simulink model "Quadcopter_close_loop"  (R2021a)
settings: Solver=ode4  StartTime=0.0  StopTime=87  FixedStep=0.001  RelTol=1e-6
values from neighbouring files (symbols this model uses):
  mean_wind = [2.72 , 1.75, -0.006]    [main_run.m]    (also in main_run_5_1.m; param_est.m = [2.72 , 1.75, .006])
  q = X(7:10)    [EKF_without_wind.m]
  r = linspace(floor(nr*0.01)/nr,1,nr)    [main_run.m]    (also in main_run_5_1.m)
  w1 = w(1)    [EKF_without_wind.m]
  x0 = [0,0,0,1,0,0,0,-P.mean_wind,0,0,0]    [main_run.m]    (also in main_run_5_1.m)
  xref = [1,1,-8,1,0,0,0,-P.mean_wind]    [main_run.m]    (also in main_run_5_1.m)
undefined symbols (not defined in the file or in its folder): HDBK, MIL, Moderate, P, u1, v1
libraries: simulink x1, aerolibwind2 x1
(part 3 of 5)

== matlab function Quadcopter_close_loop/Estimator/Estimator/EKF_quadcopter ==
  data: sensor input; y output; P parameter
function y = EKF_quadcopter(sensor,P)
%% parameters 
ts = 0.01;
m = P.m;
g = P.g;
rho = P.rho;
D = P.D;
A_gr = [0;0;g];
B_i = P.B_i;

param = cell(1,6);
param{1} = A_gr;
param{2} = m;
param{3} = rho;
param{4} = D;
param{5} = ts;
param{6} = B_i;

Q_est = P.Q_est;
R_est = P.R_est;
X0_hat = P.X0_hat;
EKF_P0 = P.EKF_P0;
%% IEKF
    persistent k P_cov X
    if isempty(k)
        k = 1;
        X = zeros(13,1);
        [X,P_cov] = EKF(X0_hat,EKF_P0,Q_est,R_est,param,sensor,k);
    end
    k = k+1;
    
    [X,P_cov] = EKF(X,P_cov,Q_est,R_est,param,sensor,k);
    
quat = X(7:10);  
eul = quat2eul(quat')';
eul([1 3]) = eul([3 1]);
X_est = [X(1:6);eul;X(11:13)];
% Asma: Dynamics states: pos, quaternion, velocity, wind? Rearranged the dynamics so that it goes into contoller correctly 

% X_est=[X(1:3); X(7:10); X(4:6); X(11:13)];

y=X_est;
end

function [X_k1,P_k1] = EKF(X,P,Q,R,param,sensor,iter)
% Performs one loop of the SP-EKF.
% Pre-Observer is of the form:
%   Xhat_dot = f(Xhat) + Fr*L*E*(Y - Yhat)

% Inputs:

%   X = State mean, m_k|k-1 (nx1)
%   P = State covariance, P_k|k-1(nxn)
%   f = State dynamics, xdot = f(x,param)
%   df = 
%   dh =
%   Q = Process Noise Covariance Matrix(nxn)
%   R = Measurement Noise Covariance Matrix (mxm)
%   param = Any parameters for f
%   iter = denotes the the first loop,1=yes,0=no

% Outputs:

%   X_k1 = state at next time step
%   P_k1 = state covariance at next time step

%parameter
A_gr = param{1};
m = param{2};
rho = param{3};
D = param{4};
ts = param{5};
B_i = param{6};
b3=[0;0;1];
%sensor
% Y=[sensor{1};sensor{2};sensor{3}]; %gps+accel+B_b
% w = sensor{4};
% f_c = sensor{5};
gps = sensor(1:3);
accel = sensor(4:6);
w = sensor(7:9);
B_b = sensor(10:12);
f_c = sensor(13);

Y=[gps;accel;B_b];
U={w;f_c}; %w+f_c
%states(13*1)
x_hat=X(1:3);
vr_hat=X(4:6);
q_hat=X(7:10);
d_hat=X(11:13);

q0=q_hat(1);q1=q_hat(2);q2=q_hat(3);q3=q_hat(4);
Ln_32 = [-q1/2, -q2/2, -q3/2;
          q0/2, -q3/2,  q2/2;
          q3/2,  q0/2, -q1/2;
         -q2/2,  q1/2,  q0/2];
%Invariant frame (13x10)
Ln =@(vr_hat)[    eye(3)      zeros(3,3)    zeros(3,1) zeros(3,3);
              zeros(3,3)     hat(vr_hat)     -(1/m)*b3  zeros(3,3);
              zeros(4,3)           Ln_32    zeros(4,1) zeros(4,3);
              zeros(3,3)      zeros(3,3)    zeros(3,1)    eye(3);];
%% time update 
    X_minus_k1 = X; %dim(X)=13x1
    P_minus_k1 = P; %dim(P)=12x12
    N=10;
    for i=1:N
    X_minus_k1 = X_minus_k1 + (ts/N).*f(X,U,param);
    
    q_hat=X_minus_k1(7:10);
    q_hat=q_hat/norm(q_hat);    
    X_minus_k1(7:10)=q_hat; %normalization
    A = df(X_minus_k1,U,param);
    
    P_minus_k1 = P_minus_k1 + (ts/N).*(A*P + P*A' + Ln(vr_hat)*Q*Ln(vr_hat)');
%     P_minus_k1 = P_minus_k1 + (ts/N)*(A*P + P*A' + Q);
    end
    X_k1 = X_minus_k1;
    P_k1 = P_minus_k1;
%% measurement update 
    H= dh(X_minus_k1,U,param);
    L = P_minus_k1*H'*inv(H*P_minus_k1*H' + R);
    X_k1 = X_minus_k1 + L*(Y-h(X_minus_k1,U,param));
    q_hat=X_k1(7:10);
    q_hat=q_hat/norm(q_hat);    
    X_k1(7:10)=q_hat; %normalization
    P_k1 = (eye(13)-L*H)*P_minus_k1;
end
 
function [X_dot] = f(X,U,param)
%states
x=X(1:3);
vr=X(4:6);
q=X(7:10);
d=X(11:13);
%inputs
w=U{1};
f_c=U{2};
%parameters
A_gr = param{1};
m = param{2};
rho = param{3};
D = param{4};
B_i= param{6};
b_3=[0;0;1];
%% system dynamics
f_vr=-(1/2)*rho*D*norm(vr)*vr;
x_dot = quat_v(q,vr,0) + d;
vr_dot = cross(vr,w) + quat_v(q,A_gr,1) - (1/m)*f_c*b_3 + (1/m)*f_vr;
q_dot = (1/2)*quat_multiply(q,[0;w]);
d_dot = [0;0;0];
%% output
X_dot = [x_dot;vr_dot;q_dot;d_dot];
end

function [Y] = h(X,U,param)
%states
x=X(1:3);
vr=X(4:6);
q=X(7:10);
d=X(11:13);
%inputs
w=U{1};
f_c=U{2};
%parameters
A_gr = param{1};
m = param{2};
rho = param{3};
D = param{4};
ts = param{5};
B_i = param{6};
b_3=[0;0;1];
%%
f_vr =-(1/2)*rho*D*norm(vr)*vr;
a = - (1/m)*f_c*b_3 + (1/m)*f_vr;
B_b = quat_v(q,B_i,1);
%% ouputs
Y = [x;a;B_b];
end

function [dfdx] = df(X,U,param)
%states
x=X(1:3);
vr=X(4:6);
vr1=vr(1);vr2=vr(2);vr3=vr(3);
q=X(7:10);
d=X(11:13);
q0=q(1);q1=q(2);q2=q(3);q3=q(4);
%inputs
w=U{1};
w1=w(1);w2=w(2);w3=w(3);
f_c=U{2};
%parameters
A_gr = param{1};
g=A_gr(3);
m = param{2};
rho = param{3};
D = param{4};
B_i= param{6};
b_3=[0;0;1];

D11=D(1,1);D22=D(2,2);D33=D(3,3);

df1dx=zeros(3,3);
df1dvr = [-2*q2^2 - 2*q3^2 + 1,2*q1*q2 - 2*q0*q3,2*q0*q2 + 2*q1*q3;
           2*q0*q3 + 2*q1*q2,-2*q1^2 - 2*q3^2 + 1,2*q2*q3 - 2*q0*q1;
           2*q1*q3 - 2*q0*q2,2*q0*q1 + 2*q2*q3,-2*q1^2 - 2*q2^2+1;];
% df1dqv = [2*q2*vr2 + 2*q3*vr3, 2*q0*vr3 + 2*q1*vr2 - 4*q2*vr1, 2*q1*vr3 - 2*q0*vr2 - 4*q3*vr1;
%           2*q2*vr1 - 4*q1*vr2 - 2*q0*vr3,2*q1*vr1 + 2*q3*vr3, 2*q0*vr1 + 2*q2*vr3 - 4*q3*vr2;
%           2*q0*vr2 - 4*q1*vr3 + 2*q3*vr1, 2*q3*vr2 - 4*q2*vr3 - 2*q0*vr1,2*q1*vr1 + 2*q2*vr2;];
df1dq = [2*q2*vr3 - 2*q3*vr2,            2*q2*vr2 + 2*q3*vr3, 2*q0*vr3 + 2*q1*vr2 - 4*q2*vr1, 2*q1*vr3 - 2*q0*vr2 - 4*q3*vr1;
         2*q3*vr1 - 2*q1*vr3, 2*q2*vr1 - 4*q1*vr2 - 2*q0*vr3,            2*q1*vr1 + 2*q3*vr3, 2*q0*vr1 + 2*q2*vr3 - 4*q3*vr2;
         2*q1*vr2 - 2*q2*vr1, 2*q0*vr2 - 4*q1*vr3 + 2*q3*vr1, 2*q3*vr2 - 4*q2*vr3 - 2*q0*vr1,            2*q1*vr1 + 2*q2*vr2];
df1dd = eye(3);

df2dx = zeros(3,3);
df2dvr =[-(D11*rho*(abs(vr1)^2 + abs(vr2)^2 + abs(vr3)^2)^(1/2))/(2*m) - (D11*rho*vr1*abs(vr1)*sign(vr1))/(2*m*(abs(vr1)^2 + abs(vr2)^2 + abs(vr3)^2)^(1/2)),                                                             w3 - (D11*rho*vr1*abs(vr2)*sign(vr2))/(2*m*(abs(vr1)^2 + abs(vr2)^2 + abs(vr3)^2)^(1/2)),                                                           - w2 - (D11*rho*vr1*abs(vr3)*sign(vr3))/(2*m*(abs(vr1)^2 + abs(vr2)^2 + abs(vr3)^2)^(1/2));
                                                                  - w3 - (D22*rho*vr2*abs(vr1)*sign(vr1))/(2*m*(abs(vr1)^2 + abs(vr2)^2 + abs(vr3)^2)^(1/2)), - (D22*rho*(abs(vr1)^2 + abs(vr2)^2 + abs(vr3)^2)^(1/2))/(2*m) - (D22*rho*vr2*abs(vr2)*sign(vr2))/(2*m*(abs(vr1)^2 + abs(vr2)^2 + abs(vr3)^2)^(1/2)),                                                             w1 - (D22*rho*vr2*abs(vr3)*sign(vr3))/(2*m*(abs(vr1)^2 + abs(vr2)^2 + abs(vr3)^2)^(1/2));
                                                                    w2 - (D33*rho*vr3*abs(vr1)*sign(vr1))/(2*m*(abs(vr1)^2 + abs(vr2)^2 + abs(vr3)^2)^(1/2)),                                                           - w1 - (D33*rho*vr3*abs(vr2)*sign(vr2))/(2*m*(abs(vr1)^2 + abs(vr2)^2 + abs(vr3)^2)^(1/2)), - (D33*rho*(abs(vr1)^2 + abs(vr2)^2 + abs(vr3)^2)^(1/2))/(2*m) - (D33*rho*vr3*abs(vr3)*sign(vr3))/(2*m*(abs(vr1)^2 + abs(vr2)^2 + abs(vr3)^2)^(1/2));];
                               
% df2dqv =[(2*g*(2*q0^2*q3 + 6*q1^2*q3 + 2*q2^2*q3 + 2*q3^3 - q3))/(4*q0^2*q1^2 + 4*q0^2*q2^2 + 4*q0^2*q3^2 + 4*q1^4 + 8*q1^2*q2^2 + 8*q1^2*q3^2 - 4*q1^2 + 4*q2^4 + 8*q2^2*q3^2 - 4*q2^2 + 4*q3^4 - 4*q3^2 + 1) - (2*g*(8*q0^2*q1 + 16*q1^3 + 16*q1*q2^2 + 16*q1*q3^2 - 8*q1)*(2*q0^2*q1*q3 - q0*q2 + 2*q1^3*q3 + 2*q1*q2^2*q3 + 2*q1*q3^3 - q1*q3))/(4*q0^2*q1^2 + 4*q0^2*q2^2 + 4*q0^2*q3^2 + 4*q1^4 + 8*q1^2*q2^2 + 8*q1^2*q3^2 - 4*q1^2 + 4*q2^4 + 8*q2^2*q3^2 - 4*q2^2 + 4*q3^4 - 4*q3^2 + 1)^2,                               - (2*g*(q0 - 4*q1*q2*q3))/(4*q0^2*q1^2 + 4*q0^2*q2^2 + 4*q0^2*q3^2 + 4*q1^4 + 8*q1^2*q2^2 + 8*q1^2*q3^2 - 4*q1^2 + 4*q2^4 + 8*q2^2*q3^2 - 4*q2^2 + 4*q3^4 - 4*q3^2 + 1) - (2*g*(8*q0^2*q2 + 16*q1^2*q2 + 16*q2^3 + 16*q2*q3^2 - 8*q2)*(2*q0^2*q1*q3 - q0*q2 + 2*q1^3*q3 + 2*q1*q2^2*q3 + 2*q1*q3^3 - q1*q3))/(4*q0^2*q1^2 + 4*q0^2*q2^2 + 4*q0^2*q3^2 + 4*q1^4 + 8*q1^2*q2^2 + 8*q1^2*q3^2 - 4*q1^2 + 4*q2^4 + 8*q2^2*q3^2 - 4*q2^2 + 4*q3^4 - 4*q3^2 + 1)^2,            (2*g*(2*q0^2*q1 + 2*q1^3 + 2*q1*q2^2 + 6*q1*q3^2 - q1))/(4*q0^2*q1^2 + 4*q0^2*q2^2 + 4*q0^2*q3^2 + 4*q1^4 + 8*q1^2*q2^2 + 8*q1^2*q3^2 - 4*q1^2 + 4*q2^4 + 8*q2^2*q3^2 - 4*q2^2 + 4*q3^4 - 4*q3^2 + 1) - (2*g*(8*q0^2*q3 + 16*q1^2*q3 + 16*q2^2*q3 + 16*q3^3 - 8*q3)*(2*q0^2*q1*q3 - q0*q2 + 2*q1^3*q3 + 2*q1*q2^2*q3 + 2*q1*q3^3 - q1*q3))/(4*q0^2*q1^2 + 4*q0^2*q2^2 + 4*q0^2*q3^2 + 4*q1^4 + 8*q1^2*q2^2 + 8*q1^2*q3^2 - 4*q1^2 + 4*q2^4 + 8*q2^2*q3^2 - 4*q2^2 + 4*q3^4 - 4*q3^2 + 1)^2;
%                                         (2*g*(q0 + 4*q1*q2*q3))/(4*q0^2*q1^2 + 4*q0^2*q2^2 + 4*q0^2*q3^2 + 4*q1^4 + 8*q1^2*q2^2 + 8*q1^2*q3^2 - 4*q1^2 + 4*q2^4 + 8*q2^2*q3^2 - 4*q2^2 + 4*q3^4 - 4*q3^2 + 1) - (2*g*(8*q0^2*q1 + 16*q1^3 + 16*q1*q2^2 + 16*q1*q3^2 - 8*q1)*(2*q0^2*q2*q3 + q0*q1 + 2*q1^2*q2*q3 + 2*q2^3*q3 + 2*q2*q3^3 - q2*q3))/(4*q0^2*q1^2 + 4*q0^2*q2^2 + 4*q0^2*q3^2 + 4*q1^4 + 8*q1^2*q2^2 + 8*q1^2*q3^2 - 4*q1^2 + 4*q2^4 + 8*q2^2*q3^2 - 4*q2^2 + 4*q3^4 - 4*q3^2 + 1)^2, (2*g*(2*q0^2*q3 + 2*q1^2*q3 + 6*q2^2*q3 + 2*q3^3 - q3))/(4*q0^2*q1^2 + 4*q0^2*q2^2 + 4*q0^2*q3^2 + 4*q1^4 + 8*q1^2*q2^2 + 8*q1^2*q3^2 - 4*q1^2 + 4*q2^4 + 8*q2^2*q3^2 - 4*q2^2 + 4*q3^4 - 4*q3^2 + 1) - (2*g*(8*q0^2*q2 + 16*q1^2*q2 + 16*q2^3 + 16*q2*q3^2 - 8*q2)*(2*q0^2*q2*q3 + q0*q1 + 2*q1^2*q2*q3 + 2*q2^3*q3 + 2*q2*q3^3 - q2*q3))/(4*q0^2*q1^2 + 4*q0^2*q2^2 + 4*q0^2*q3^2 + 4*q1^4 + 8*q1^2*q2^2 + 8*q1^2*q3^2 - 4*q1^2 + 4*q2^4 + 8*q2^2*q3^2 - 4*q2^2 + 4*q3^4 - 4*q3^2 + 1)^2,            (2*g*(2*q0^2*q2 + 2*q1^2*q2 + 2*q2^3 + 6*q2*q3^2 - q2))/(4*q0^2*q1^2 + 4*q0^2*q2^2 + 4*q0^2*q3^2 + 4*q1^4 + 8*q1^2*q2^2 + 8*q1^2*q3^2 - 4*q1^2 + 4*q2^4 + 8*q2^2*q3^2 - 4*q2^2 + 4*q3^4 - 4*q3^2 + 1) - (2*g*(8*q0^2*q3 + 16*q1^2*q3 + 16*q2^2*q3 + 16*q3^3 - 8*q3)*(2*q0^2*q2*q3 + q0*q1 + 2*q1^2*q2*q3 + 2*q2^3*q3 + 2*q2*q3^3 - q2*q3))/(4*q0^2*q1^2 + 4*q0^2*q2^2 + 4*q0^2*q3^2 + 4*q1^4 + 8*q1^2*q2^2 + 8*q1^2*q3^2 - 4*q1^2 + 4*q2^4 + 8*q2^2*q3^2 - 4*q2^2 + 4*q3^4 - 4*q3^2 + 1)^2;
%                            - (g*(- 8*q1*q3^2 + 4*q1))/(4*q0^2*q1^2 + 4*q0^2*q2^2 + 4*q0^2*q3^2 + 4*q1^4 + 8*q1^2*q2^2 + 8*q1^2*q3^2 - 4*q1^2 + 4*q2^4 + 8*q2^2*q3^2 - 4*q2^2 + 4*q3^4 - 4*q3^2 + 1) - (g*(8*q0^2*q1 + 16*q1^3 + 16*q1*q2^2 + 16*q1*q3^2 - 8*q1)*(4*q0^2*q3^2 + 4*q1^2*q3^2 - 2*q1^2 + 4*q2^2*q3^2 - 2*q2^2 + 4*q3^4 - 4*q3^2 + 1))/(4*q0^2*q1^2 + 4*q0^2*q2^2 + 4*q0^2*q3^2 + 4*q1^4 + 8*q1^2*q2^2 + 8*q1^2*q3^2 - 4*q1^2 + 4*q2^4 + 8*q2^2*q3^2 - 4*q2^2 + 4*q3^4 - 4*q3^2 + 1)^2,                    - (g*(- 8*q2*q3^2 + 4*q2))/(4*q0^2*q1^2 + 4*q0^2*q2^2 + 4*q0^2*q3^2 + 4*q1^4 + 8*q1^2*q2^2 + 8*q1^2*q3^2 - 4*q1^2 + 4*q2^4 + 8*q2^2*q3^2 - 4*q2^2 + 4*q3^4 - 4*q3^2 + 1) - (g*(8*q0^2*q2 + 16*q1^2*q2 + 16*q2^3 + 16*q2*q3^2 - 8*q2)*(4*q0^2*q3^2 + 4*q1^2*q3^2 - 2*q1^2 + 4*q2^2*q3^2 - 2*q2^2 + 4*q3^4 - 4*q3^2 + 1))/(4*q0^2*q1^2 + 4*q0^2*q2^2 + 4*q0^2*q3^2 + 4*q1^4 + 8*q1^2*q2^2 + 8*q1^2*q3^2 - 4*q1^2 + 4*q2^4 + 8*q2^2*q3^2 - 4*q2^2 + 4*q3^4 - 4*q3^2 + 1)^2, (g*(8*q0^2*q3 + 8*q1^2*q3 + 8*q2^2*q3 + 16*q3^3 - 8*q3))/(4*q0^2*q1^2 + 4*q0^2*q2^2 + 4*q0^2*q3^2 + 4*q1^4 + 8*q1^2*q2^2 + 8*q1^2*q3^2 - 4*q1^2 + 4*q2^4 + 8*q2^2*q3^2 - 4*q2^2 + 4*q3^4 - 4*q3^2 + 1) - (g*(8*q0^2*q3 + 16*q1^2*q3 + 16*q2^2*q3 + 16*q3^3 - 8*q3)*(4*q0^2*q3^2 + 4*q1^2*q3^2 - 2*q1^2 + 4*q2^2*q3^2 - 2*q2^2 + 4*q3^4 - 4*q3^2 + 1))/(4*q0^2*q1^2 + 4*q0^2*q2^2 + 4*q0^2*q3^2 + 4*q1^4 + 8*q1^2*q2^2 + 8*q1^2*q3^2 - 4*q1^2 + 4*q2^4 + 8*q2^2*q3^2 - 4*q2^2 + 4*q3^4 - 4*q3^2 + 1)^2];
df2dq=[- (2*g*(q2 - 4*q0*q1*q3))/(4*q0^2*q1^2 + 4*q0^2*q2^2 + 4*q0^2*q3^2 + 4*q1^4 + 8*q1^2*q2^2 + 8*q1^2*q3^2 - 4*q1^2 + 4*q2^4 + 8*q2^2*q3^2 - 4*q2^2 + 4*q3^4 - 4*q3^2 + 1) - (2*g*(8*q0*q1^2 + 8*q0*q2^2 + 8*q0*q3^2)*(2*q0^2*q1*q3 - q0*q2 + 2*q1^3*q3 + 2*q1*q2^2*q3 + 2*q1*q3^3 - q1*q3))/(4*q0^2*q1^2 + 4*q0^2*q2^2 + 4*q0^2*q3^2 + 4*q1^4 + 8*q1^2*q2^2 + 8*q1^2*q3^2 - 4*q1^2 + 4*q2^4 + 8*q2^2*q3^2 - 4*q2^2 + 4*q3^4 - 4*q3^2 + 1)^2, (2*g*(2*q0^2*q3 + 6*q1^2*q3 + 2*q2^2*q3 + 2*q3^3 - q3))/(4*q0^2*q1^2 + 4*q0^2*q2^2 + 4*q0^2*q3^2 + 4*q1^4 + 8*q1^2*q2^2 + 8*q1^2*q3^2 - 4*q1^2 + 4*q2^4 + 8*q2^2*q3^2 - 4*q2^2 + 4*q3^4 - 4*q3^2 + 1) - (2*g*(8*q0^2*q1 + 16*q1^3 + 16*q1*q2^2 + 16*q1*q3^2 - 8*q1)*(2*q0^2*q1*q3 - q0*q2 + 2*q1^3*q3 + 2*q1*q2^2*q3 + 2*q1*q3^3 - q1*q3))/(4*q0^2*q1^2 + 4*q0^2*q2^2 + 4*q0^2*q3^2 + 4*q1^4 + 8*q1^2*q2^2 + 8*q1^2*q3^2 - 4*q1^2 + 4*q2^4 + 8*q2^2*q3^2 - 4*q2^2 + 4*q3^4 - 4*q3^2 + 1)^2,                               - (2*g*(q0 - 4*q1*q2*q3))/(4*q0^2*q1^2 + 4*q0^2*q2^2 + 4*q0^2*q3^2 + 4*q1^4 + 8*q1^2*q2^2 + 8*q1^2*q3^2 - 4*q1^2 + 4*q2^4 + 8*q2^2*q3^2 - 4*q2^2 + 4*q3^4 - 4*q3^2 + 1) - (2*g*(8*q0^2*q2 + 16*q1^2*q2 + 16*q2^3 + 16*q2*q3^2 - 8*q2)*(2*q0^2*q1*q3 - q0*q2 + 2*q1^3*q3 + 2*q1*q2^2*q3 + 2*q1*q3^3 - q1*q3))/(4*q0^2*q1^2 + 4*q0^2*q2^2 + 4*q0^2*q3^2 + 4*q1^4 + 8*q1^2*q2^2 + 8*q1^2*q3^2 - 4*q1^2 + 4*q2^4 + 8*q2^2*q3^2 - 4*q2^2 + 4*q3^4 - 4*q3^2 + 1)^2,            (2*g*(2*q0^2*q1 + 2*q1^3 + 2*q1*q2^2 + 6*q1*q3^2 - q1))/(4*q0^2*q1^2 + 4*q0^2*q2^2 + 4*q0^2*q3^2 + 4*q1^4 + 8*q1^2*q2^2 + 8*q1^2*q3^2 - 4*q1^2 + 4*q2^4 + 8*q2^2*q3^2 - 4*q2^2 + 4*q3^4 - 4*q3^2 + 1) - (2*g*(8*q0^2*q3 + 16*q1^2*q3 + 16*q2^2*q3 + 16*q3^3 - 8*q3)*(2*q0^2*q1*q3 - q0*q2 + 2*q1^3*q3 + 2*q1*q2^2*q3 + 2*q1*q3^3 - q1*q3))/(4*q0^2*q1^2 + 4*q0^2*q2^2 + 4*q0^2*q3^2 + 4*q1^4 + 8*q1^2*q2^2 + 8*q1^2*q3^2 - 4*q1^2 + 4*q2^4 + 8*q2^2*q3^2 - 4*q2^2 + 4*q3^4 - 4*q3^2 + 1)^2;
       (2*g*(q1 + 4*q0*q2*q3))/(4*q0^2*q1^2 + 4*q0^2*q2^2 + 4*q0^2*q3^2 + 4*q1^4 + 8*q1^2*q2^2 + 8*q1^2*q3^2 - 4*q1^2 + 4*q2^4 + 8*q2^2*q3^2 - 4*q2^2 + 4*q3^4 - 4*q3^2 + 1) - (2*g*(8*q0*q1^2 + 8*q0*q2^2 + 8*q0*q3^2)*(2*q0^2*q2*q3 + q0*q1 + 2*q1^2*q2*q3 + 2*q2^3*q3 + 2*q2*q3^3 - q2*q3))/(4*q0^2*q1^2 + 4*q0^2*q2^2 + 4*q0^2*q3^2 + 4*q1^4 + 8*q1^2*q2^2 + 8*q1^2*q3^2 - 4*q1^2 + 4*q2^4 + 8*q2^2*q3^2 - 4*q2^2 + 4*q3^4 - 4*q3^2 + 1)^2,                                 (2*g*(q0 + 4*q1*q2*q3))/(4*q0^2*q1^2 + 4*q0^2*q2^2 + 4*q0^2*q3^2 + 4*q1^4 + 8*q1^2*q2^2 + 8*q1^2*q3^2 - 4*q1^2 + 4*q2^4 + 8*q2^2*q3^2 - 4*q2^2 + 4*q3^4 - 4*q3^2 + 1) - (2*g*(8*q0^2*q1 + 16*q1^3 + 16*q1*q2^2 + 16*q1*q3^2 - 8*q1)*(2*q0^2*q2*q3 + q0*q1 + 2*q1^2*q2*q3 + 2*q2^3*q3 + 2*q2*q3^3 - q2*q3))/(4*q0^2*q1^2 + 4*q0^2*q2^2 + 4*q0^2*q3^2 + 4*q1^4 + 8*q1^2*q2^2 + 8*q1^2*q3^2 - 4*q1^2 + 4*q2^4 + 8*q2^2*q3^2 - 4*q2^2 + 4*q3^4 - 4*q3^2 + 1)^2, (2*g*(2*q0^2*q3 + 2*q1^2*q3 + 6*q2^2*q3 + 2*q3^3 - q3))/(4*q0^2*q1^2 + 4*q0^2*q2^2 + 4*q0^2*q3^2 + 4*q1^4 + 8*q1^2*q2^2 + 8*q1^2*q3^2 - 4*q1^2 + 4*q2^4 + 8*q2^2*q3^2 - 4*q2^2 + 4*q3^4 - 4*q3^2 + 1) - (2*g*(8*q0^2*q2 + 16*q1^2*q2 + 16*q2^3 + 16*q2*q3^2 - 8*q2)*(2*q0^2*q2*q3 + q0*q1 + 2*q1^2*q2*q3 + 2*q2^3*q3 + 2*q2*q3^3 - q2*q3))/(4*q0^2*q1^2 + 4*q0^2*q2^2 + 4*q0^2*q3^2 + 4*q1^4 + 8*q1^2*q2^2 + 8*q1^2*q3^2 - 4*q1^2 + 4*q2^4 + 8*q2^2*q3^2 - 4*q2^2 + 4*q3^4 - 4*q3^2 + 1)^2,            (2*g*(2*q0^2*q2 + 2*q1^2*q2 + 2*q2^3 + 6*q2*q3^2 - q2))/(4*q0^2*q1^2 + 4*q0^2*q2^2 + 4*q0^2*q3^2 + 4*q1^4 + 8*q1^2*q2^2 + 8*q1^2*q3^2 - 4*q1^2 + 4*q2^4 + 8*q2^2*q3^2 - 4*q2^2 + 4*q3^4 - 4*q3^2 + 1) - (2*g*(8*q0^2*q3 + 16*q1^2*q3 + 16*q2^2*q3 + 16*q3^3 - 8*q3)*(2*q0^2*q2*q3 + q0*q1 + 2*q1^2*q2*q3 + 2*q2^3*q3 + 2*q2*q3^3 - q2*q3))/(4*q0^2*q1^2 + 4*q0^2*q2^2 + 4*q0^2*q3^2 + 4*q1^4 + 8*q1^2*q2^2 + 8*q1^2*q3^2 - 4*q1^2 + 4*q2^4 + 8*q2^2*q3^2 - 4*q2^2 + 4*q3^4 - 4*q3^2 + 1)^2;
        (8*g*q0*q3^2)/(4*q0^2*q1^2 + 4*q0^2*q2^2 + 4*q0^2*q3^2 + 4*q1^4 + 8*q1^2*q2^2 + 8*q1^2*q3^2 - 4*q1^2 + 4*q2^4 + 8*q2^2*q3^2 - 4*q2^2 + 4*q3^4 - 4*q3^2 + 1) - (g*(8*q0*q1^2 + 8*q0*q2^2 + 8*q0*q3^2)*(4*q0^2*q3^2 + 4*q1^2*q3^2 - 2*q1^2 + 4*q2^2*q3^2 - 2*q2^2 + 4*q3^4 - 4*q3^2 + 1))/(4*q0^2*q1^2 + 4*q0^2*q2^2 + 4*q0^2*q3^2 + 4*q1^4 + 8*q1^2*q2^2 + 8*q1^2*q3^2 - 4*q1^2 + 4*q2^4 + 8*q2^2*q3^2 - 4*q2^2 + 4*q3^4 - 4*q3^2 + 1)^2,                    - (g*(- 8*q1*q3^2 + 4*q1))/(4*q0^2*q1^2 + 4*q0^2*q2^2 + 4*q0^2*q3^2 + 4*q1^4 + 8*q1^2*q2^2 + 8*q1^2*q3^2 - 4*q1^2 + 4*q2^4 + 8*q2^2*q3^2 - 4*q2^2 + 4*q3^4 - 4*q3^2 + 1) - (g*(8*q0^2*q1 + 16*q1^3 + 16*q1*q2^2 + 16*q1*q3^2 - 8*q1)*(4*q0^2*q3^2 + 4*q1^2*q3^2 - 2*q1^2 + 4*q2^2*q3^2 - 2*q2^2 + 4*q3^4 - 4*q3^2 + 1))/(4*q0^2*q1^2 + 4*q0^2*q2^2 + 4*q0^2*q3^2 + 4*q1^4 + 8*q1^2*q2^2 + 8*q1^2*q3^2 - 4*q1^2 + 4*q2^4 + 8*q2^2*q3^2 - 4*q2^2 + 4*q3^4 - 4*q3^2 + 1)^2,                    - (g*(- 8*q2*q3^2 + 4*q2))/(4*q0^2*q1^2 + 4*q0^2*q2^2 + 4*q0^2*q3^2 + 4*q1^4 + 8*q1^2*q2^2 + 8*q1^2*q3^2 - 4*q1^2 + 4*q2^4 + 8*q2^2*q3^2 - 4*q2^2 + 4*q3^4 - 4*q3^2 + 1) - (g*(8*q0^2*q2 + 16*q1^2*q2 + 16*q2^3 + 16*q2*q3^2 - 8*q2)*(4*q0^2*q3^2 + 4*q1^2*q3^2 - 2*q1^2 + 4*q2^2*q3^2 - 2*q2^2 + 4*q3^4 - 4*q3^2 + 1))/(4*q0^2*q1^2 + 4*q0^2*q2^2 + 4*q0^2*q3^2 + 4*q1^4 + 8*q1^2*q2^2 + 8*q1^2*q3^2 - 4*q1^2 + 4*q2^4 + 8*q2^2*q3^2 - 4*q2^2 + 4*q3^4 - 4*q3^2 + 1)^2, (g*(8*q0^2*q3 + 8*q1^2*q3 + 8*q2^2*q3 + 16*q3^3 - 8*q3))/(4*q0^2*q1^2 + 4*q0^2*q2^2 + 4*q0^2*q3^2 + 4*q1^4 + 8*q1^2*q2^2 + 8*q1^2*q3^2 - 4*q1^2 + 4*q2^4 + 8*q2^2*q3^2 - 4*q2^2 + 4*q3^4 - 4*q3^2 + 1) - (g*(8*q0^2*q3 + 16*q1^2*q3 + 16*q2^2*q3 + 16*q3^3 - 8*q3)*(4*q0^2*q3^2 + 4*q1^2*q3^2 - 2*q1^2 + 4*q2^2*q3^2 - 2*q2^2 + 4*q3^4 - 4*q3^2 + 1))/(4*q0^2*q1^2 + 4*q0^2*q2^2 + 4*q0^2*q3^2 + 4*q1^4 + 8*q1^2*q2^2 + 8*q1^2*q3^2 - 4*q1^2 + 4*q2^4 + 8*q2^2*q3^2 - 4*q2^2 + 4*q3^4 - 4*q3^2 + 1)^2];

df2dd = zeros(3,3);

df3dx = zeros(4,3);
df3dvr = zeros(4,3);
% df3dqv = -hat(w);
df3dq=[   0, -w1/2, -w2/2, -w3/2;
       w1/2,     0,  w3/2, -w2/2;
       w2/2, -w3/2,     0,  w1/2;
       w3/2,  w2/2, -w1/2,     0];
df3dd = zeros(4,3);

df4dx = zeros(3,3);
df4dvr = zeros(3,3);
% df4dqv = zeros(3,3);
df4dq = zeros(3,4);
df4dd = zeros(3,3);

dfdx = [df1dx df1dvr df1dq df1dd;
        df2dx df2dvr df2dq df2dd;
        df3dx df3dvr df3dq df3dd;
        df4dx df4dvr df4dq df4dd]; 
end

function [dhdX] = dh(X,U,param) 
%states
x=X(1:3);
vr=X(4:6);
q=X(7:10);
d=X(11:13);

vr1=vr(1);vr2=vr(2);vr3=vr(3);
q0=q(1);q1=q(2);q2=q(3);q3=q(4);
%inputs
w=U{1};
f_c=U{2};
%parameters
A_gr = param{1};
m = param{2};
rho = param{3};
D = param{4};
ts = param{5};
B_i= param{6};
b_3=[0;0;1];

B_i1 = B_i(1);B_i2 = B_i(2);B_i3 = B_i(3);
D11=D(1,1);D22=D(2,2);D33=D(3,3);
%%
dh1dx = eye(3);
dh1dvr= zeros(3,3);
% dh1dqv= zeros(3,3);
dh1dq= zeros(3,4);
dh1dd= zeros(3,3);

dh2dx  = zeros(3,3);
dh2dvr = [-(D11*rho*(abs(vr1)^2 + abs(vr2)^2 + abs(vr3)^2)^(1/2))/(2*m) - (D11*rho*vr1*abs(vr1)*sign(vr1))/(2*m*(abs(vr1)^2 + abs(vr2)^2 + abs(vr3)^2)^(1/2)),                                                                 -(D11*rho*vr1*abs(vr2)*sign(vr2))/(2*m*(abs(vr1)^2 + abs(vr2)^2 + abs(vr3)^2)^(1/2)),                                                                 -(D11*rho*vr1*abs(vr3)*sign(vr3))/(2*m*(abs(vr1)^2 + abs(vr2)^2 + abs(vr3)^2)^(1/2));
                                                                        -(D22*rho*vr2*abs(vr1)*sign(vr1))/(2*m*(abs(vr1)^2 + abs(vr2)^2 + abs(vr3)^2)^(1/2)), - (D22*rho*(abs(vr1)^2 + abs(vr2)^2 + abs(vr3)^2)^(1/2))/(2*m) - (D22*rho*vr2*abs(vr2)*sign(vr2))/(2*m*(abs(vr1)^2 + abs(vr2)^2 + abs(vr3)^2)^(1/2)),                                                                 -(D22*rho*vr2*abs(vr3)*sign(vr3))/(2*m*(abs(vr1)^2 + abs(vr2)^2 + abs(vr3)^2)^(1/2));
                                                                        -(D33*rho*vr3*abs(vr1)*sign(vr1))/(2*m*(abs(vr1)^2 + abs(vr2)^2 + abs(vr3)^2)^(1/2)),                                                                 -(D33*rho*vr3*abs(vr2)*sign(vr2))/(2*m*(abs(vr1)^2 + abs(vr2)^2 + abs(vr3)^2)^(1/2)), - (D33*rho*(abs(vr1)^2 + abs(vr2)^2 + abs(vr3)^2)^(1/2))/(2*m) - (D33*rho*vr3*abs(vr3)*sign(vr3))/(2*m*(abs(vr1)^2 + abs(vr2)^2 + abs(vr3)^2)^(1/2))];

% dh2dqv = zeros(3,3);
dh2dq = zeros(3,4);
dh2dd  = zeros(3,3);

dh3dx = zeros(3,3);
dh3dvr= zeros(3,3);
% dh3dqv= [(2*B_i2*(2*q0^2*q2 + 6*q1^2*q2 + 2*q2^3 + 2*q2*q3^2 - q2))/(4*q0^2*q1^2 + 4*q0^2*q2^2 + 4*q0^2*q3^2 + 4*q1^4 + 8*q1^2*q2^2 + 8*q1^2*q3^2 - 4*q1^2 + 4*q2^4 + 8*q2^2*q3^2 - 4*q2^2 + 4*q3^4 - 4*q3^2 + 1) + (2*B_i3*(2*q0^2*q3 + 6*q1^2*q3 + 2*q2^2*q3 + 2*q3^3 - q3))/(4*q0^2*q1^2 + 4*q0^2*q2^2 + 4*q0^2*q3^2 + 4*q1^4 + 8*q1^2*q2^2 + 8*q1^2*q3^2 - 4*q1^2 + 4*q2^4 + 8*q2^2*q3^2 - 4*q2^2 + 4*q3^4 - 4*q3^2 + 1) + (B_i1*(8*q0^2*q1 + 16*q1^3 + 8*q1*q2^2 + 8*q1*q3^2 - 8*q1))/(4*q0^2*q1^2 + 4*q0^2*q2^2 + 4*q0^2*q3^2 + 4*q1^4 + 8*q1^2*q2^2 + 8*q1^2*q3^2 - 4*q1^2 + 4*q2^4 + 8*q2^2*q3^2 - 4*q2^2 + 4*q3^4 - 4*q3^2 + 1) - (2*B_i2*(8*q0^2*q1 + 16*q1^3 + 16*q1*q2^2 + 16*q1*q3^2 - 8*q1)*(2*q0^2*q1*q2 + q0*q3 + 2*q1^3*q2 + 2*q1*q2^3 + 2*q1*q2*q3^2 - q1*q2))/(4*q0^2*q1^2 + 4*q0^2*q2^2 + 4*q0^2*q3^2 + 4*q1^4 + 8*q1^2*q2^2 + 8*q1^2*q3^2 - 4*q1^2 + 4*q2^4 + 8*q2^2*q3^2 - 4*q2^2 + 4*q3^4 - 4*q3^2 + 1)^2 - (2*B_i3*(8*q0^2*q1 + 16*q1^3 + 16*q1*q2^2 + 16*q1*q3^2 - 8*q1)*(2*q0^2*q1*q3 - q0*q2 + 2*q1^3*q3 + 2*q1*q2^2*q3 + 2*q1*q3^3 - q1*q3))/(4*q0^2*q1^2 + 4*q0^2*q2^2 + 4*q0^2*q3^2 + 4*q1^4 + 8*q1^2*q2^2 + 8*q1^2*q3^2 - 4*q1^2 + 4*q2^4 + 8*q2^2*q3^2 - 4*q2^2 + 4*q3^4 - 4*q3^2 + 1)^2 - (B_i1*(8*q0^2*q1 + 16*q1^3 + 16*q1*q2^2 + 16*q1*q3^2 - 8*q1)*(4*q0^2*q1^2 + 4*q1^4 + 4*q1^2*q2^2 + 4*q1^2*q3^2 - 4*q1^2 - 2*q2^2 - 2*q3^2 + 1))/(4*q0^2*q1^2 + 4*q0^2*q2^2 + 4*q0^2*q3^2 + 4*q1^4 + 8*q1^2*q2^2 + 8*q1^2*q3^2 - 4*q1^2 + 4*q2^4 + 8*q2^2*q3^2 - 4*q2^2 + 4*q3^4 - 4*q3^2 + 1)^2,                                                                 (2*B_i2*(2*q0^2*q1 + 2*q1^3 + 6*q1*q2^2 + 2*q1*q3^2 - q1))/(4*q0^2*q1^2 + 4*q0^2*q2^2 + 4*q0^2*q3^2 + 4*q1^4 + 8*q1^2*q2^2 + 8*q1^2*q3^2 - 4*q1^2 + 4*q2^4 + 8*q2^2*q3^2 - 4*q2^2 + 4*q3^4 - 4*q3^2 + 1) - (B_i1*(- 8*q2*q1^2 + 4*q2))/(4*q0^2*q1^2 + 4*q0^2*q2^2 + 4*q0^2*q3^2 + 4*q1^4 + 8*q1^2*q2^2 + 8*q1^2*q3^2 - 4*q1^2 + 4*q2^4 + 8*q2^2*q3^2 - 4*q2^2 + 4*q3^4 - 4*q3^2 + 1) - (2*B_i3*(q0 - 4*q1*q2*q3))/(4*q0^2*q1^2 + 4*q0^2*q2^2 + 4*q0^2*q3^2 + 4*q1^4 + 8*q1^2*q2^2 + 8*q1^2*q3^2 - 4*q1^2 + 4*q2^4 + 8*q2^2*q3^2 - 4*q2^2 + 4*q3^4 - 4*q3^2 + 1) - (2*B_i2*(8*q0^2*q2 + 16*q1^2*q2 + 16*q2^3 + 16*q2*q3^2 - 8*q2)*(2*q0^2*q1*q2 + q0*q3 + 2*q1^3*q2 + 2*q1*q2^3 + 2*q1*q2*q3^2 - q1*q2))/(4*q0^2*q1^2 + 4*q0^2*q2^2 + 4*q0^2*q3^2 + 4*q1^4 + 8*q1^2*q2^2 + 8*q1^2*q3^2 - 4*q1^2 + 4*q2^4 + 8*q2^2*q3^2 - 4*q2^2 + 4*q3^4 - 4*q3^2 + 1)^2 - (2*B_i3*(8*q0^2*q2 + 16*q1^2*q2 + 16*q2^3 + 16*q2*q3^2 - 8*q2)*(2*q0^2*q1*q3 - q0*q2 + 2*q1^3*q3 + 2*q1*q2^2*q3 + 2*q1*q3^3 - q1*q3))/(4*q0^2*q1^2 + 4*q0^2*q2^2 + 4*q0^2*q3^2 + 4*q1^4 + 8*q1^2*q2^2 + 8*q1^2*q3^2 - 4*q1^2 + 4*q2^4 + 8*q2^2*q3^2 - 4*q2^2 + 4*q3^4 - 4*q3^2 + 1)^2 - (B_i1*(8*q0^2*q2 + 16*q1^2*q2 + 16*q2^3 + 16*q2*q3^2 - 8*q2)*(4*q0^2*q1^2 + 4*q1^4 + 4*q1^2*q2^2 + 4*q1^2*q3^2 - 4*q1^2 - 2*q2^2 - 2*q3^2 + 1))/(4*q0^2*q1^2 + 4*q0^2*q2^2 + 4*q0^2*q3^2 + 4*q1^4 + 8*q1^2*q2^2 + 8*q1^2*q3^2 - 4*q1^2 + 4*q2^4 + 8*q2^2*q3^2 - 4*q2^2 + 4*q3^4 - 4*q3^2 + 1)^2,                                                                 (2*B_i2*(q0 + 4*q1*q2*q3))/(4*q0^2*q1^2 + 4*q0^2*q2^2 + 4*q0^2*q3^2 + 4*q1^4 + 8*q1^2*q2^2 + 8*q1^2*q3^2 - 4*q1^2 + 4*q2^4 + 8*q2^2*q3^2 - 4*q2^2 + 4*q3^4 - 4*q3^2 + 1) - (B_i1*(- 8*q3*q1^2 + 4*q3))/(4*q0^2*q1^2 + 4*q0^2*q2^2 + 4*q0^2*q3^2 + 4*q1^4 + 8*q1^2*q2^2 + 8*q1^2*q3^2 - 4*q1^2 + 4*q2^4 + 8*q2^2*q3^2 - 4*q2^2 + 4*q3^4 - 4*q3^2 + 1) + (2*B_i3*(2*q0^2*q1 + 2*q1^3 + 2*q1*q2^2 + 6*q1*q3^2 - q1))/(4*q0^2*q1^2 + 4*q0^2*q2^2 + 4*q0^2*q3^2 + 4*q1^4 + 8*q1^2*q2^2 + 8*q1^2*q3^2 - 4*q1^2 + 4*q2^4 + 8*q2^2*q3^2 - 4*q2^2 + 4*q3^4 - 4*q3^2 + 1) - (2*B_i2*(8*q0^2*q3 + 16*q1^2*q3 + 16*q2^2*q3 + 16*q3^3 - 8*q3)*(2*q0^2*q1*q2 + q0*q3 + 2*q1^3*q2 + 2*q1*q2^3 + 2*q1*q2*q3^2 - q1*q2))/(4*q0^2*q1^2 + 4*q0^2*q2^2 + 4*q0^2*q3^2 + 4*q1^4 + 8*q1^2*q2^2 + 8*q1^2*q3^2 - 4*q1^2 + 4*q2^4 + 8*q2^2*q3^2 - 4*q2^2 + 4*q3^4 - 4*q3^2 + 1)^2 - (2*B_i3*(8*q0^2*q3 + 16*q1^2*q3 + 16*q2^2*q3 + 16*q3^3 - 8*q3)*(2*q0^2*q1*q3 - q0*q2 + 2*q1^3*q3 + 2*q1*q2^2*q3 + 2*q1*q3^3 - q1*q3))/(4*q0^2*q1^2 + 4*q0^2*q2^2 + 4*q0^2*q3^2 + 4*q1^4 + 8*q1^2*q2^2 + 8*q1^2*q3^2 - 4*q1^2 + 4*q2^4 + 8*q2^2*q3^2 - 4*q2^2 + 4*q3^4 - 4*q3^2 + 1)^2 - (B_i1*(8*q0^2*q3 + 16*q1^2*q3 + 16*q2^2*q3 + 16*q3^3 - 8*q3)*(4*q0^2*q1^2 + 4*q1^4 + 4*q1^2*q2^2 + 4*q1^2*q3^2 - 4*q1^2 - 2*q2^2 - 2*q3^2 + 1))/(4*q0^2*q1^2 + 4*q0^2*q2^2 + 4*q0^2*q3^2 + 4*q1^4 + 8*q1^2*q2^2 + 8*q1^2*q3^2 - 4*q1^2 + 4*q2^4 + 8*q2^2*q3^2 - 4*q2^2 + 4*q3^4 - 4*q3^2 + 1)^2;
%                                                                 (2*B_i3*(q0 + 4*q1*q2*q3))/(4*q0^2*q1^2 + 4*q0^2*q2^2 + 4*q0^2*q3^2 + 4*q1^4 + 8*q1^2*q2^2 + 8*q1^2*q3^2 - 4*q1^2 + 4*q2^4 + 8*q2^2*q3^2 - 4*q2^2 + 4*q3^4 - 4*q3^2 + 1) - (B_i2*(- 8*q1*q2^2 + 4*q1))/(4*q0^2*q1^2 + 4*q0^2*q2^2 + 4*q0^2*q3^2 + 4*q1^4 + 8*q1^2*q2^2 + 8*q1^2*q3^2 - 4*q1^2 + 4*q2^4 + 8*q2^2*q3^2 - 4*q2^2 + 4*q3^4 - 4*q3^2 + 1) + (2*B_i1*(2*q0^2*q2 + 6*q1^2*q2 + 2*q2^3 + 2*q2*q3^2 - q2))/(4*q0^2*q1^2 + 4*q0^2*q2^2 + 4*q0^2*q3^2 + 4*q1^4 + 8*q1^2*q2^2 + 8*q1^2*q3^2 - 4*q1^2 + 4*q2^4 + 8*q2^2*q3^2 - 4*q2^2 + 4*q3^4 - 4*q3^2 + 1) - (2*B_i1*(8*q0^2*q1 + 16*q1^3 + 16*q1*q2^2 + 16*q1*q3^2 - 8*q1)*(2*q0^2*q1*q2 - q0*q3 + 2*q1^3*q2 + 2*q1*q2^3 + 2*q1*q2*q3^2 - q1*q2))/(4*q0^2*q1^2 + 4*q0^2*q2^2 + 4*q0^2*q3^2 + 4*q1^4 + 8*q1^2*q2^2 + 8*q1^2*q3^2 - 4*q1^2 + 4*q2^4 + 8*q2^2*q3^2 - 4*q2^2 + 4*q3^4 - 4*q3^2 + 1)^2 - (2*B_i3*(8*q0^2*q1 + 16*q1^3 + 16*q1*q2^2 + 16*q1*q3^2 - 8*q1)*(2*q0^2*q2*q3 + q0*q1 + 2*q1^2*q2*q3 + 2*q2^3*q3 + 2*q2*q3^3 - q2*q3))/(4*q0^2*q1^2 + 4*q0^2*q2^2 + 4*q0^2*q3^2 + 4*q1^4 + 8*q1^2*q2^2 + 8*q1^2*q3^2 - 4*q1^2 + 4*q2^4 + 8*q2^2*q3^2 - 4*q2^2 + 4*q3^4 - 4*q3^2 + 1)^2 - (B_i2*(8*q0^2*q1 + 16*q1^3 + 16*q1*q2^2 + 16*q1*q3^2 - 8*q1)*(4*q0^2*q2^2 + 4*q1^2*q2^2 - 2*q1^2 + 4*q2^4 + 4*q2^2*q3^2 - 4*q2^2 - 2*q3^2 + 1))/(4*q0^2*q1^2 + 4*q0^2*q2^2 + 4*q0^2*q3^2 + 4*q1^4 + 8*q1^2*q2^2 + 8*q1^2*q3^2 - 4*q1^2 + 4*q2^4 + 8*q2^2*q3^2 - 4*q2^2 + 4*q3^4 - 4*q3^2 + 1)^2, (2*B_i1*(2*q0^2*q1 + 2*q1^3 + 6*q1*q2^2 + 2*q1*q3^2 - q1))/(4*q0^2*q1^2 + 4*q0^2*q2^2 + 4*q0^2*q3^2 + 4*q1^4 + 8*q1^2*q2^2 + 8*q1^2*q3^2 - 4*q1^2 + 4*q2^4 + 8*q2^2*q3^2 - 4*q2^2 + 4*q3^4 - 4*q3^2 + 1) + (2*B_i3*(2*q0^2*q3 + 2*q1^2*q3 + 6*q2^2*q3 + 2*q3^3 - q3))/(4*q0^2*q1^2 + 4*q0^2*q2^2 + 4*q0^2*q3^2 + 4*q1^4 + 8*q1^2*q2^2 + 8*q1^2*q3^2 - 4*q1^2 + 4*q2^4 + 8*q2^2*q3^2 - 4*q2^2 + 4*q3^4 - 4*q3^2 + 1) + (B_i2*(8*q0^2*q2 + 8*q1^2*q2 + 16*q2^3 + 8*q2*q3^2 - 8*q2))/(4*q0^2*q1^2 + 4*q0^2*q2^2 + 4*q0^2*q3^2 + 4*q1^4 + 8*q1^2*q2^2 + 8*q1^2*q3^2 - 4*q1^2 + 4*q2^4 + 8*q2^2*q3^2 - 4*q2^2 + 4*q3^4 - 4*q3^2 + 1) - (2*B_i1*(8*q0^2*q2 + 16*q1^2*q2 + 16*q2^3 + 16*q2*q3^2 - 8*q2)*(2*q0^2*q1*q2 - q0*q3 + 2*q1^3*q2 + 2*q1*q2^3 + 2*q1*q2*q3^2 - q1*q2))/(4*q0^2*q1^2 + 4*q0^2*q2^2 + 4*q0^2*q3^2 + 4*q1^4 + 8*q1^2*q2^2 + 8*q1^2*q3^2 - 4*q1^2 + 4*q2^4 + 8*q2^2*q3^2 - 4*q2^2 + 4*q3^4 - 4*q3^2 + 1)^2 - (2*B_i3*(8*q0^2*q2 + 16*q1^2*q2 + 16*q2^3 + 16*q2*q3^2 - 8*q2)*(2*q0^2*q2*q3 + q0*q1 + 2*q1^2*q2*q3 + 2*q2^3*q3 + 2*q2*q3^3 - q2*q3))/(4*q0^2*q1^2 + 4*q0^2*q2^2 + 4*q0^2*q3^2 + 4*q1^4 + 8*q1^2*q2^2 + 8*q1^2*q3^2 - 4*q1^2 + 4*q2^4 + 8*q2^2*q3^2 - 4*q2^2 + 4*q3^4 - 4*q3^2 + 1)^2 - (B_i2*(8*q0^2*q2 + 16*q1^2*q2 + 16*q2^3 + 16*q2*q3^2 - 8*q2)*(4*q0^2*q2^2 + 4*q1^2*q2^2 - 2*q1^2 + 4*q2^4 + 4*q2^2*q3^2 - 4*q2^2 - 2*q3^2 + 1))/(4*q0^2*q1^2 + 4*q0^2*q2^2 + 4*q0^2*q3^2 + 4*q1^4 + 8*q1^2*q2^2 + 8*q1^2*q3^2 - 4*q1^2 + 4*q2^4 + 8*q2^2*q3^2 - 4*q2^2 + 4*q3^4 - 4*q3^2 + 1)^2,                                                                 (2*B_i3*(2*q0^2*q2 + 2*q1^2*q2 + 2*q2^3 + 6*q2*q3^2 - q2))/(4*q0^2*q1^2 + 4*q0^2*q2^2 + 4*q0^2*q3^2 + 4*q1^4 + 8*q1^2*q2^2 + 8*q1^2*q3^2 - 4*q1^2 + 4*q2^4 + 8*q2^2*q3^2 - 4*q2^2 + 4*q3^4 - 4*q3^2 + 1) - (B_i2*(- 8*q3*q2^2 + 4*q3))/(4*q0^2*q1^2 + 4*q0^2*q2^2 + 4*q0^2*q3^2 + 4*q1^4 + 8*q1^2*q2^2 + 8*q1^2*q3^2 - 4*q1^2 + 4*q2^4 + 8*q2^2*q3^2 - 4*q2^2 + 4*q3^4 - 4*q3^2 + 1) - (2*B_i1*(q0 - 4*q1*q2*q3))/(4*q0^2*q1^2 + 4*q0^2*q2^2 + 4*q0^2*q3^2 + 4*q1^4 + 8*q1^2*q2^2 + 8*q1^2*q3^2 - 4*q1^2 + 4*q2^4 + 8*q2^2*q3^2 - 4*q2^2 + 4*q3^4 - 4*q3^2 + 1) - (2*B_i1*(8*q0^2*q3 + 16*q1^2*q3 + 16*q2^2*q3 + 16*q3^3 - 8*q3)*(2*q0^2*q1*q2 - q0*q3 + 2*q1^3*q2 + 2*q1*q2^3 + 2*q1*q2*q3^2 - q1*q2))/(4*q0^2*q1^2 + 4*q0^2*q2^2 + 4*q0^2*q3^2 + 4*q1^4 + 8*q1^2*q2^2 + 8*q1^2*q3^2 - 4*q1^2 + 4*q2^4 + 8*q2^2*q3^2 - 4*q2^2 + 4*q3^4 - 4*q3^2 + 1)^2 - (2*B_i3*(8*q0^2*q3 + 16*q1^2*q3 + 16*q2^2*q3 + 16*q3^3 - 8*q3)*(2*q0^2*q2*q3 + q0*q1 + 2*q1^2*q2*q3 + 2*q2^3*q3 + 2*q2*q3^3 - q2*q3))/(4*q0^2*q1^2 + 4*q0^2*q2^2 + 4*q0^2*q3^2 + 4*q1^4 + 8*q1^2*q2^2 + 8*q1^2*q3^2 - 4*q1^2 + 4*q2^4 + 8*q2^2*q3^2 - 4*q2^2 + 4*q3^4 - 4*q3^2 + 1)^2 - (B_i2*(8*q0^2*q3 + 16*q1^2*q3 + 16*q2^2*q3 + 16*q3^3 - 8*q3)*(4*q0^2*q2^2 + 4*q1^2*q2^2 - 2*q1^2 + 4*q2^4 + 4*q2^2*q3^2 - 4*q2^2 - 2*q3^2 + 1))/(4*q0^2*q1^2 + 4*q0^2*q2^2 + 4*q0^2*q3^2 + 4*q1^4 + 8*q1^2*q2^2 + 8*q1^2*q3^2 - 4*q1^2 + 4*q2^4 + 8*q2^2*q3^2 - 4*q2^2 + 4*q3^4 - 4*q3^2 + 1)^2;
%                                                                 (2*B_i1*(2*q0^2*q3 + 6*q1^2*q3 + 2*q2^2*q3 + 2*q3^3 - q3))/(4*q0^2*q1^2 + 4*q0^2*q2^2 + 4*q0^2*q3^2 + 4*q1^4 + 8*q1^2*q2^2 + 8*q1^2*q3^2 - 4*q1^2 + 4*q2^4 + 8*q2^2*q3^2 - 4*q2^2 + 4*q3^4 - 4*q3^2 + 1) - (B_i3*(- 8*q1*q3^2 + 4*q1))/(4*q0^2*q1^2 + 4*q0^2*q2^2 + 4*q0^2*q3^2 + 4*q1^4 + 8*q1^2*q2^2 + 8*q1^2*q3^2 - 4*q1^2 + 4*q2^4 + 8*q2^2*q3^2 - 4*q2^2 + 4*q3^4 - 4*q3^2 + 1) - (2*B_i2*(q0 - 4*q1*q2*q3))/(4*q0^2*q1^2 + 4*q0^2*q2^2 + 4*q0^2*q3^2 + 4*q1^4 + 8*q1^2*q2^2 + 8*q1^2*q3^2 - 4*q1^2 + 4*q2^4 + 8*q2^2*q3^2 - 4*q2^2 + 4*q3^4 - 4*q3^2 + 1) - (2*B_i1*(8*q0^2*q1 + 16*q1^3 + 16*q1*q2^2 + 16*q1*q3^2 - 8*q1)*(2*q0^2*q1*q3 + q0*q2 + 2*q1^3*q3 + 2*q1*q2^2*q3 + 2*q1*q3^3 - q1*q3))/(4*q0^2*q1^2 + 4*q0^2*q2^2 + 4*q0^2*q3^2 + 4*q1^4 + 8*q1^2*q2^2 + 8*q1^2*q3^2 - 4*q1^2 + 4*q2^4 + 8*q2^2*q3^2 - 4*q2^2 + 4*q3^4 - 4*q3^2 + 1)^2 - (2*B_i2*(8*q0^2*q1 + 16*q1^3 + 16*q1*q2^2 + 16*q1*q3^2 - 8*q1)*(2*q0^2*q2*q3 - q0*q1 + 2*q1^2*q2*q3 + 2*q2^3*q3 + 2*q2*q3^3 - q2*q3))/(4*q0^2*q1^2 + 4*q0^2*q2^2 + 4*q0^2*q3^2 + 4*q1^4 + 8*q1^2*q2^2 + 8*q1^2*q3^2 - 4*q1^2 + 4*q2^4 + 8*q2^2*q3^2 - 4*q2^2 + 4*q3^4 - 4*q3^2 + 1)^2 - (B_i3*(8*q0^2*q1 + 16*q1^3 + 16*q1*q2^2 + 16*q1*q3^2 - 8*q1)*(4*q0^2*q3^2 + 4*q1^2*q3^2 - 2*q1^2 + 4*q2^2*q3^2 - 2*q2^2 + 4*q3^4 - 4*q3^2 + 1))/(4*q0^2*q1^2 + 4*q0^2*q2^2 + 4*q0^2*q3^2 + 4*q1^4 + 8*q1^2*q2^2 + 8*q1^2*q3^2 - 4*q1^2 + 4*q2^4 + 8*q2^2*q3^2 - 4*q2^2 + 4*q3^4 - 4*q3^2 + 1)^2,                                                                 (2*B_i1*(q0 + 4*q1*q2*q3))/(4*q0^2*q1^2 + 4*q0^2*q2^2 + 4*q0^2*q3^2 + 4*q1^4 + 8*q1^2*q2^2 + 8*q1^2*q3^2 - 4*q1^2 + 4*q2^4 + 8*q2^2*q3^2 - 4*q2^2 + 4*q3^4 - 4*q3^2 + 1) - (B_i3*(- 8*q2*q3^2 + 4*q2))/(4*q0^2*q1^2 + 4*q0^2*q2^2 + 4*q0^2*q3^2 + 4*q1^4 + 8*q1^2*q2^2 + 8*q1^2*q3^2 - 4*q1^2 + 4*q2^4 + 8*q2^2*q3^2 - 4*q2^2 + 4*q3^4 - 4*q3^2 + 1) + (2*B_i2*(2*q0^2*q3 + 2*q1^2*q3 + 6*q2^2*q3 + 2*q3^3 - q3))/(4*q0^2*q1^2 + 4*q0^2*q2^2 + 4*q0^2*q3^2 + 4*q1^4 + 8*q1^2*q2^2 + 8*q1^2*q3^2 - 4*q1^2 + 4*q2^4 + 8*q2^2*q3^2 - 4*q2^2 + 4*q3^4 - 4*q3^2 + 1) - (2*B_i1*(8*q0^2*q2 + 16*q1^2*q2 + 16*q2^3 + 16*q2*q3^2 - 8*q2)*(2*q0^2*q1*q3 + q0*q2 + 2*q1^3*q3 + 2*q1*q2^2*q3 + 2*q1*q3^3 - q1*q3))/(4*q0^2*q1^2 + 4*q0^2*q2^2 + 4*q0^2*q3^2 + 4*q1^4 + 8*q1^2*q2^2 + 8*q1^2*q3^2 - 4*q1^2 + 4*q2^4 + 8*q2^2*q3^2 - 4*q2^2 + 4*q3^4 - 4*q3^2 + 1)^2 - (2*B_i2*(8*q0^2*q2 + 16*q1^2*q2 + 16*q2^3 + 16*q2*q3^2 - 8*q2)*(2*q0^2*q2*q3 - q0*q1 + 2*q1^2*q2*q3 + 2*q2^3*q3 + 2*q2*q3^3 - q2*q3))/(4*q0^2*q1^2 + 4*q0^2*q2^2 + 4*q0^2*q3^2 + 4*q1^4 + 8*q1^2*q2^2 + 8*q1^2*q3^2 - 4*q1^2 + 4*q2^4 + 8*q2^2*q3^2 - 4*q2^2 + 4*q3^4 - 4*q3^2 + 1)^2 - (B_i3*(8*q0^2*q2 + 16*q1^2*q2 + 16*q2^3 + 16*q2*q3^2 - 8*q2)*(4*q0^2*q3^2 + 4*q1^2*q3^2 - 2*q1^2 + 4*q2^2*q3^2 - 2*q2^2 + 4*q3^4 - 4*q3^2 + 1))/(4*q0^2*q1^2 + 4*q0^2*q2^2 + 4*q0^2*q3^2 + 4*q1^4 + 8*q1^2*q2^2 + 8*q1^2*q3^2 - 4*q1^2 + 4*q2^4 + 8*q2^2*q3^2 - 4*q2^2 + 4*q3^4 - 4*q3^2 + 1)^2, (2*B_i1*(2*q0^2*q1 + 2*q1^3 + 2*q1*q2^2 + 6*q1*q3^2 - q1))/(4*q0^2*q1^2 + 4*q0^2*q2^2 + 4*q0^2*q3^2 + 4*q1^4 + 8*q1^2*q2^2 + 8*q1^2*q3^2 - 4*q1^2 + 4*q2^4 + 8*q2^2*q3^2 - 4*q2^2 + 4*q3^4 - 4*q3^2 + 1) + (2*B_i2*(2*q0^2*q2 + 2*q1^2*q2 + 2*q2^3 + 6*q2*q3^2 - q2))/(4*q0^2*q1^2 + 4*q0^2*q2^2 + 4*q0^2*q3^2 + 4*q1^4 + 8*q1^2*q2^2 + 8*q1^2*q3^2 - 4*q1^2 + 4*q2^4 + 8*q2^2*q3^2 - 4*q2^2 + 4*q3^4 - 4*q3^2 + 1) + (B_i3*(8*q0^2*q3 + 8*q1^2*q3 + 8*q2^2*q3 + 16*q3^3 - 8*q3))/(4*q0^2*q1^2 + 4*q0^2*q2^2 + 4*q0^2*q3^2 + 4*q1^4 + 8*q1^2*q2^2 + 8*q1^2*q3^2 - 4*q1^2 + 4*q2^4 + 8*q2^2*q3^2 - 4*q2^2 + 4*q3^4 - 4*q3^2 + 1) - (2*B_i1*(8*q0^2*q3 + 16*q1^2*q3 + 16*q2^2*q3 + 16*q3^3 - 8*q3)*(2*q0^2*q1*q3 + q0*q2 + 2*q1^3*q3 + 2*q1*q2^2*q3 + 2*q1*q3^3 - q1*q3))/(4*q0^2*q1^2 + 4*q0^2*q2^2 + 4*q0^2*q3^2 + 4*q1^4 + 8*q1^2*q2^2 + 8*q1^2*q3^2 - 4*q1^2 + 4*q2^4 + 8*q2^2*q3^2 - 4*q2^2 + 4*q3^4 - 4*q3^2 + 1)^2 - (2*B_i2*(8*q0^2*q3 + 16*q1^2*q3 + 16*q2^2*q3 + 16*q3^3 - 8*q3)*(2*q0^2*q2*q3 - q0*q1 + 2*q1^2*q2*q3 + 2*q2^3*q3 + 2*q2*q3^3 - q2*q3))/(4*q0^2*q1^2 + 4*q0^2*q2^2 + 4*q0^2*q3^2 + 4*q1^4 + 8*q1^2*q2^2 + 8*q1^2*q3^2 - 4*q1^2 + 4*q2^4 + 8*q2^2*q3^2 - 4*q2^2 + 4*q3^4 - 4*q3^2 + 1)^2 - (B_i3*(8*q0^2*q3 + 16*q1^2*q3 + 16*q2^2*q3 + 16*q3^3 - 8*q3)*(4*q0^2*q3^2 + 4*q1^2*q3^2 - 2*q1^2 + 4*q2^2*q3^2 - 2*q2^2 + 4*q3^4 - 4*q3^2 + 1))/(4*q0^2*q1^2 + 4*q0^2*q2^2 + 4*q0^2*q3^2 + 4*q1^4 + 8*q1^2*q2^2 + 8*q1^2*q3^2 - 4*q1^2 + 4*q2^4 + 8*q2^2*q3^2 - 4*q2^2 + 4*q3^4 - 4*q3^2 + 1)^2];
dh3dq = [(2*B_i2*(q3 + 4*q0*q1*q2))/(4*q0^2*q1^2 + 4*q0^2*q2^2 + 4*q0^2*q3^2 + 4*q1^4 + 8*q1^2*q2^2 + 8*q1^2*q3^2 - 4*q1^2 + 4*q2^4 + 8*q2^2*q3^2 - 4*q2^2 + 4*q3^4 - 4*q3^2 + 1) - (2*B_i3*(q2 - 4*q0*q1*q3))/(4*q0^2*q1^2 + 4*q0^2*q2^2 + 4*q0^2*q3^2 + 4*q1^4 + 8*q1^2*q2^2 + 8*q1^2*q3^2 - 4*q1^2 + 4*q2^4 + 8*q2^2*q3^2 - 4*q2^2 + 4*q3^4 - 4*q3^2 + 1) - (2*B_i2*(8*q0*q1^2 + 8*q0*q2^2 + 8*q0*q3^2)*(2*q0^2*q1*q2 + q0*q3 + 2*q1^3*q2 + 2*q1*q2^3 + 2*q1*q2*q3^2 - q1*q2))/(4*q0^2*q1^2 + 4*q0^2*q2^2 + 4*q0^2*q3^2 + 4*q1^4 + 8*q1^2*q2^2 + 8*q1^2*q3^2 - 4*q1^2 + 4*q2^4 + 8*q2^2*q3^2 - 4*q2^2 + 4*q3^4 - 4*q3^2 + 1)^2 - (2*B_i3*(8*q0*q1^2 + 8*q0*q2^2 + 8*q0*q3^2)*(2*q0^2*q1*q3 - q0*q2 + 2*q1^3*q3 + 2*q1*q2^2*q3 + 2*q1*q3^3 - q1*q3))/(4*q0^2*q1^2 + 4*q0^2*q2^2 + 4*q0^2*q3^2 + 4*q1^4 + 8*q1^2*q2^2 + 8*q1^2*q3^2 - 4*q1^2 + 4*q2^4 + 8*q2^2*q3^2 - 4*q2^2 + 4*q3^4 - 4*q3^2 + 1)^2 + (8*B_i1*q0*q1^2)/(4*q0^2*q1^2 + 4*q0^2*q2^2 + 4*q0^2*q3^2 + 4*q1^4 + 8*q1^2*q2^2 + 8*q1^2*q3^2 - 4*q1^2 + 4*q2^4 + 8*q2^2*q3^2 - 4*q2^2 + 4*q3^4 - 4*q3^2 + 1) - (B_i1*(8*q0*q1^2 + 8*q0*q2^2 + 8*q0*q3^2)*(4*q0^2*q1^2 + 4*q1^4 + 4*q1^2*q2^2 + 4*q1^2*q3^2 - 4*q1^2 - 2*q2^2 - 2*q3^2 + 1))/(4*q0^2*q1^2 + 4*q0^2*q2^2 + 4*q0^2*q3^2 + 4*q1^4 + 8*q1^2*q2^2 + 8*q1^2*q3^2 - 4*q1^2 + 4*q2^4 + 8*q2^2*q3^2 - 4*q2^2 + 4*q3^4 - 4*q3^2 + 1)^2, (2*B_i2*(2*q0^2*q2 + 6*q1^2*q2 + 2*q2^3 + 2*q2*q3^2 - q2))/(4*q0^2*q1^2 + 4*q0^2*q2^2 + 4*q0^2*q3^2 + 4*q1^4 + 8*q1^2*q2^2 + 8*q1^2*q3^2 - 4*q1^2 + 4*q2^4 + 8*q2^2*q3^2 - 4*q2^2 + 4*q3^4 - 4*q3^2 + 1) + (2*B_i3*(2*q0^2*q3 + 6*q1^2*q3 + 2*q2^2*q3 + 2*q3^3 - q3))/(4*q0^2*q1^2 + 4*q0^2*q2^2 + 4*q0^2*q3^2 + 4*q1^4 + 8*q1^2*q2^2 + 8*q1^2*q3^2 - 4*q1^2 + 4*q2^4 + 8*q2^2*q3^2 - 4*q2^2 + 4*q3^4 - 4*q3^2 + 1) + (B_i1*(8*q0^2*q1 + 16*q1^3 + 8*q1*q2^2 + 8*q1*q3^2 - 8*q1))/(4*q0^2*q1^2 + 4*q0^2*q2^2 + 4*q0^2*q3^2 + 4*q1^4 + 8*q1^2*q2^2 + 8*q1^2*q3^2 - 4*q1^2 + 4*q2^4 + 8*q2^2*q3^2 - 4*q2^2 + 4*q3^4 - 4*q3^2 + 1) - (2*B_i2*(8*q0^2*q1 + 16*q1^3 + 16*q1*q2^2 + 16*q1*q3^2 - 8*q1)*(2*q0^2*q1*q2 + q0*q3 + 2*q1^3*q2 + 2*q1*q2^3 + 2*q1*q2*q3^2 - q1*q2))/(4*q0^2*q1^2 + 4*q0^2*q2^2 + 4*q0^2*q3^2 + 4*q1^4 + 8*q1^2*q2^2 + 8*q1^2*q3^2 - 4*q1^2 + 4*q2^4 + 8*q2^2*q3^2 - 4*q2^2 + 4*q3^4 - 4*q3^2 + 1)^2 - (2*B_i3*(8*q0^2*q1 + 16*q1^3 + 16*q1*q2^2 + 16*q1*q3^2 - 8*q1)*(2*q0^2*q1*q3 - q0*q2 + 2*q1^3*q3 + 2*q1*q2^2*q3 + 2*q1*q3^3 - q1*q3))/(4*q0^2*q1^2 + 4*q0^2*q2^2 + 4*q0^2*q3^2 + 4*q1^4 + 8*q1^2*q2^2 + 8*q1^2*q3^2 - 4*q1^2 + 4*q2^4 + 8*q2^2*q3^2 - 4*q2^2 + 4*q3^4 - 4*q3^2 + 1)^2 - (B_i1*(8*q0^2*q1 + 16*q1^3 + 16*q1*q2^2 + 16*q1*q3^2 - 8*q1)*(4*q0^2*q1^2 + 4*q1^4 + 4*q1^2*q2^2 + 4*q1^2*q3^2 - 4*q1^2 - 2*q2^2 - 2*q3^2 + 1))/(4*q0^2*q1^2 + 4*q0^2*q2^2 + 4*q0^2*q3^2 + 4*q1^4 + 8*q1^2*q2^2 + 8*q1^2*q3^2 - 4*q1^2 + 4*q2^4 + 8*q2^2*q3^2 - 4*q2^2 + 4*q3^4 - 4*q3^2 + 1)^2,                                                                 (2*B_i2*(2*q0^2*q1 + 2*q1^3 + 6*q1*q2^2 + 2*q1*q3^2 - q1))/(4*q0^2*q1^2 + 4*q0^2*q2^2 + 4*q0^2*q3^2 + 4*q1^4 + 8*q1^2*q2^2 + 8*q1^2*q3^2 - 4*q1^2 + 4*q2^4 + 8*q2^2*q3^2 - 4*q2^2 + 4*q3^4 - 4*q3^2 + 1) - (B_i1*(- 8*q2*q1^2 + 4*q2))/(4*q0^2*q1^2 + 4*q0^2*q2^2 + 4*q0^2*q3^2 + 4*q1^4 + 8*q1^2*q2^2 + 8*q1^2*q3^2 - 4*q1^2 + 4*q2^4 + 8*q2^2*q3^2 - 4*q2^2 + 4*q3^4 - 4*q3^2 + 1) - (2*B_i3*(q0 - 4*q1*q2*q3))/(4*q0^2*q1^2 + 4*q0^2*q2^2 + 4*q0^2*q3^2 + 4*q1^4 + 8*q1^2*q2^2 + 8*q1^2*q3^2 - 4*q1^2 + 4*q2^4 + 8*q2^2*q3^2 - 4*q2^2 + 4*q3^4 - 4*q3^2 + 1) - (2*B_i2*(8*q0^2*q2 + 16*q1^2*q2 + 16*q2^3 + 16*q2*q3^2 - 8*q2)*(2*q0^2*q1*q2 + q0*q3 + 2*q1^3*q2 + 2*q1*q2^3 + 2*q1*q2*q3^2 - q1*q2))/(4*q0^2*q1^2 + 4*q0^2*q2^2 + 4*q0^2*q3^2 + 4*q1^4 + 8*q1^2*q2^2 + 8*q1^2*q3^2 - 4*q1^2 + 4*q2^4 + 8*q2^2*q3^2 - 4*q2^2 + 4*q3^4 - 4*q3^2 + 1)^2 - (2*B_i3*(8*q0^2*q2 + 16*q1^2*q2 + 16*q2^3 + 16*q2*q3^2 - 8*q2)*(2*q0^2*q1*q3 - q0*q2 + 2*q1^3*q3 + 2*q1*q2^2*q3 + 2*q1*q3^3 - q1*q3))/(4*q0^2*q1^2 + 4*q0^2*q2^2 + 4*q0^2*q3^2 + 4*q1^4 + 8*q1^2*q2^2 + 8*q1^2*q3^2 - 4*q1^2 + 4*q2^4 + 8*q2^2*q3^2 - 4*q2^2 + 4*q3^4 - 4*q3^2 + 1)^2 - (B_i1*(8*q0^2*q2 + 16*q1^2*q2 + 16*q2^3 + 16*q2*q3^2 - 8*q2)*(4*q0^2*q1^2 + 4*q1^4 + 4*q1^2*q2^2 + 4*q1^2*q3^2 - 4*q1^2 - 2*q2^2 - 2*q3^2 + 1))/(4*q0^2*q1^2 + 4*q0^2*q2^2 + 4*q0^2*q3^2 + 4*q1^4 + 8*q1^2*q2^2 + 8*q1^2*q3^2 - 4*q1^2 + 4*q2^4 + 8*q2^2*q3^2 - 4*q2^2 + 4*q3^4 - 4*q3^2 + 1)^2,                                                                 (2*B_i2*(q0 + 4*q1*q2*q3))/(4*q0^2*q1^2 + 4*q0^2*q2^2 + 4*q0^2*q3^2 + 4*q1^4 + 8*q1^2*q2^2 + 8*q1^2*q3^2 - 4*q1^2 + 4*q2^4 + 8*q2^2*q3^2 - 4*q2^2 + 4*q3^4 - 4*q3^2 + 1) - (B_i1*(- 8*q3*q1^2 + 4*q3))/(4*q0^2*q1^2 + 4*q0^2*q2^2 + 4*q0^2*q3^2 + 4*q1^4 + 8*q1^2*q2^2 + 8*q1^2*q3^2 - 4*q1^2 + 4*q2^4 + 8*q2^2*q3^2 - 4*q2^2 + 4*q3^4 - 4*q3^2 + 1) + (2*B_i3*(2*q0^2*q1 + 2*q1^3 + 2*q1*q2^2 + 6*q1*q3^2 - q1))/(4*q0^2*q1^2 + 4*q0^2*q2^2 + 4*q0^2*q3^2 + 4*q1^4 + 8*q1^2*q2^2 + 8*q1^2*q3^2 - 4*q1^2 + 4*q2^4 + 8*q2^2*q3^2 - 4*q2^2 + 4*q3^4 - 4*q3^2 + 1) - (2*B_i2*(8*q0^2*q3 + 16*q1^2*q3 + 16*q2^2*q3 + 16*q3^3 - 8*q3)*(2*q0^2*q1*q2 + q0*q3 + 2*q1^3*q2 + 2*q1*q2^3 + 2*q1*q2*q3^2 - q1*q2))/(4*q0^2*q1^2 + 4*q0^2*q2^2 + 4*q0^2*q3^2 + 4*q1^4 + 8*q1^2*q2^2 + 8*q1^2*q3^2 - 4*q1^2 + 4*q2^4 + 8*q2^2*q3^2 - 4*q2^2 + 4*q3^4 - 4*q3^2 + 1)^2 - (2*B_i3*(8*q0^2*q3 + 16*q1^2*q3 + 16*q2^2*q3 + 16*q3^3 - 8*q3)*(2*q0^2*q1*q3 - q0*q2 + 2*q1^3*q3 + 2*q1*q2^2*q3 + 2*q1*q3^3 - q1*q3))/(4*q0^2*q1^2 + 4*q0^2*q2^2 + 4*q0^2*q3^2 + 4*q1^4 + 8*q1^2*q2^2 + 8*q1^2*q3^2 - 4*q1^2 + 4*q2^4 + 8*q2^2*q3^2 - 4*q2^2 + 4*q3^4 - 4*q3^2 + 1)^2 - (B_i1*(8*q0^2*q3 + 16*q1^2*q3 + 16*q2^2*q3 + 16*q3^3 - 8*q3)*(4*q0^2*q1^2 + 4*q1^4 + 4*q1^2*q2^2 + 4*q1^2*q3^2 - 4*q1^2 - 2*q2^2 - 2*q3^2 + 1))/(4*q0^2*q1^2 + 4*q0^2*q2^2 + 4*q0^2*q3^2 + 4*q1^4 + 8*q1^2*q2^2 + 8*q1^2*q3^2 - 4*q1^2 + 4*q2^4 + 8*q2^2*q3^2 - 4*q2^2 + 4*q3^4 - 4*q3^2 + 1)^2;
        (2*B_i3*(q1 + 4*q0*q2*q3))/(4*q0^2*q1^2 + 4*q0^2*q2^2 + 4*q0^2*q3^2 + 4*q1^4 + 8*q1^2*q2^2 + 8*q1^2*q3^2 - 4*q1^2 + 4*q2^4 + 8*q2^2*q3^2 - 4*q2^2 + 4*q3^4 - 4*q3^2 + 1) - (2*B_i1*(q3 - 4*q0*q1*q2))/(4*q0^2*q1^2 + 4*q0^2*q2^2 + 4*q0^2*q3^2 + 4*q1^4 + 8*q1^2*q2^2 + 8*q1^2*q3^2 - 4*q1^2 + 4*q2^4 + 8*q2^2*q3^2 - 4*q2^2 + 4*q3^4 - 4*q3^2 + 1) - (2*B_i1*(8*q0*q1^2 + 8*q0*q2^2 + 8*q0*q3^2)*(2*q0^2*q1*q2 - q0*q3 + 2*q1^3*q2 + 2*q1*q2^3 + 2*q1*q2*q3^2 - q1*q2))/(4*q0^2*q1^2 + 4*q0^2*q2^2 + 4*q0^2*q3^2 + 4*q1^4 + 8*q1^2*q2^2 + 8*q1^2*q3^2 - 4*q1^2 + 4*q2^4 + 8*q2^2*q3^2 - 4*q2^2 + 4*q3^4 - 4*q3^2 + 1)^2 - (2*B_i3*(8*q0*q1^2 + 8*q0*q2^2 + 8*q0*q3^2)*(2*q0^2*q2*q3 + q0*q1 + 2*q1^2*q2*q3 + 2*q2^3*q3 + 2*q2*q3^3 - q2*q3))/(4*q0^2*q1^2 + 4*q0^2*q2^2 + 4*q0^2*q3^2 + 4*q1^4 + 8*q1^2*q2^2 + 8*q1^2*q3^2 - 4*q1^2 + 4*q2^4 + 8*q2^2*q3^2 - 4*q2^2 + 4*q3^4 - 4*q3^2 + 1)^2 + (8*B_i2*q0*q2^2)/(4*q0^2*q1^2 + 4*q0^2*q2^2 + 4*q0^2*q3^2 + 4*q1^4 + 8*q1^2*q2^2 + 8*q1^2*q3^2 - 4*q1^2 + 4*q2^4 + 8*q2^2*q3^2 - 4*q2^2 + 4*q3^4 - 4*q3^2 + 1) - (B_i2*(8*q0*q1^2 + 8*q0*q2^2 + 8*q0*q3^2)*(4*q0^2*q2^2 + 4*q1^2*q2^2 - 2*q1^2 + 4*q2^4 + 4*q2^2*q3^2 - 4*q2^2 - 2*q3^2 + 1))/(4*q0^2*q1^2 + 4*q0^2*q2^2 + 4*q0^2*q3^2 + 4*q1^4 + 8*q1^2*q2^2 + 8*q1^2*q3^2 - 4*q1^2 + 4*q2^4 + 8*q2^2*q3^2 - 4*q2^2 + 4*q3^4 - 4*q3^2 + 1)^2,                                                                 (2*B_i3*(q0 + 4*q1*q2*q3))/(4*q0^2*q1^2 + 4*q0^2*q2^2 + 4*q0^2*q3^2 + 4*q1^4 + 8*q1^2*q2^2 + 8*q1^2*q3^2 - 4*q1^2 + 4*q2^4 + 8*q2^2*q3^2 - 4*q2^2 + 4*q3^4 - 4*q3^2 + 1) - (B_i2*(- 8*q1*q2^2 + 4*q1))/(4*q0^2*q1^2 + 4*q0^2*q2^2 + 4*q0^2*q3^2 + 4*q1^4 + 8*q1^2*q2^2 + 8*q1^2*q3^2 - 4*q1^2 + 4*q2^4 + 8*q2^2*q3^2 - 4*q2^2 + 4*q3^4 - 4*q3^2 + 1) + (2*B_i1*(2*q0^2*q2 + 6*q1^2*q2 + 2*q2^3 + 2*q2*q3^2 - q2))/(4*q0^2*q1^2 + 4*q0^2*q2^2 + 4*q0^2*q3^2 + 4*q1^4 + 8*q1^2*q2^2 + 8*q1^2*q3^2 - 4*q1^2 + 4*q2^4 + 8*q2^2*q3^2 - 4*q2^2 + 4*q3^4 - 4*q3^2 + 1) - (2*B_i1*(8*q0^2*q1 + 16*q1^3 + 16*q1*q2^2 + 16*q1*q3^2 - 8*q1)*(2*q0^2*q1*q2 - q0*q3 + 2*q1^3*q2 + 2*q1*q2^3 + 2*q1*q2*q3^2 - q1*q2))/(4*q0^2*q1^2 + 4*q0^2*q2^2 + 4*q0^2*q3^2 + 4*q1^4 + 8*q1^2*q2^2 + 8*q1^2*q3^2 - 4*q1^2 + 4*q2^4 + 8*q2^2*q3^2 - 4*q2^2 + 4*q3^4 - 4*q3^2 + 1)^2 - (2*B_i3*(8*q0^2*q1 + 16*q1^3 + 16*q1*q2^2 + 16*q1*q3^2 - 8*q1)*(2*q0^2*q2*q3 + q0*q1 + 2*q1^2*q2*q3 + 2*q2^3*q3 + 2*q2*q3^3 - q2*q3))/(4*q0^2*q1^2 + 4*q0^2*q2^2 + 4*q0^2*q3^2 + 4*q1^4 + 8*q1^2*q2^2 + 8*q1^2*q3^2 - 4*q1^2 + 4*q2^4 + 8*q2^2*q3^2 - 4*q2^2 + 4*q3^4 - 4*q3^2 + 1)^2 - (B_i2*(8*q0^2*q1 + 16*q1^3 + 16*q1*q2^2 + 16*q1*q3^2 - 8*q1)*(4*q0^2*q2^2 + 4*q1^2*q2^2 - 2*q1^2 + 4*q2^4 + 4*q2^2*q3^2 - 4*q2^2 - 2*q3^2 + 1))/(4*q0^2*q1^2 + 4*q0^2*q2^2 + 4*q0^2*q3^2 + 4*q1^4 + 8*q1^2*q2^2 + 8*q1^2*q3^2 - 4*q1^2 + 4*q2^4 + 8*q2^2*q3^2 - 4*q2^2 + 4*q3^4 - 4*q3^2 + 1)^2, (2*B_i1*(2*q0^2*q1 + 2*q1^3 + 6*q1*q2^2 + 2*q1*q3^2 - q1))/(4*q0^2*q1^2 + 4*q0^2*q2^2 + 4*q0^2*q3^2 + 4*q1^4 + 8*q1^2*q2^2 + 8*q1^2*q3^2 - 4*q1^2 + 4*q2^4 + 8*q2^2*q3^2 - 4*q2^2 + 4*q3^4 - 4*q3^2 + 1) + (2*B_i3*(2*q0^2*q3 + 2*q1^2*q3 + 6*q2^2*q3 + 2*q3^3 - q3))/(4*q0^2*q1^2 + 4*q0^2*q2^2 + 4*q0^2*q3^2 + 4*q1^4 + 8*q1^2*q2^2 + 8*q1^2*q3^2 - 4*q1^2 + 4*q2^4 + 8*q2^2*q3^2 - 4*q2^2 + 4*q3^4 - 4*q3^2 + 1) + (B_i2*(8*q0^2*q2 + 8*q1^2*q2 + 16*q2^3 + 8*q2*q3^2 - 8*q2))/(4*q0^2*q1^2 + 4*q0^2*q2^2 + 4*q0^2*q3^2 + 4*q1^4 + 8*q1^2*q2^2 + 8*q1^2*q3^2 - 4*q1^2 + 4*q2^4 + 8*q2^2*q3^2 - 4*q2^2 + 4*q3^4 - 4*q3^2 + 1) - (2*B_i1*(8*q0^2*q2 + 16*q1^2*q2 + 16*q2^3 + 16*q2*q3^2 - 8*q2)*(2*q0^2*q1*q2 - q0*q3 + 2*q1^3*q2 + 2*q1*q2^3 + 2*q1*q2*q3^2 - q1*q2))/(4*q0^2*q1^2 + 4*q0^2*q2^2 + 4*q0^2*q3^2 + 4*q1^4 + 8*q1^2*q2^2 + 8*q1^2*q3^2 - 4*q1^2 + 4*q2^4 + 8*q2^2*q3^2 - 4*q2^2 + 4*q3^4 - 4*q3^2 + 1)^2 - (2*B_i3*(8*q0^2*q2 + 16*q1^2*q2 + 16*q2^3 + 16*q2*q3^2 - 8*q2)*(2*q0^2*q2*q3 + q0*q1 + 2*q1^2*q2*q3 + 2*q2^3*q3 + 2*q2*q3^3 - q2*q3))/(4*q0^2*q1^2 + 4*q0^2*q2^2 + 4*q0^2*q3^2 + 4*q1^4 + 8*q1^2*q2^2 + 8*q1^2*q3^2 - 4*q1^2 + 4*q2^4 + 8*q2^2*q3^2 - 4*q2^2 + 4*q3^4 - 4*q3^2 + 1)^2 - (B_i2*(8*q0^2*q2 + 16*q1^2*q2 + 16*q2^3 + 16*q2*q3^2 - 8*q2)*(4*q0^2*q2^2 + 4*q1^2*q2^2 - 2*q1^2 + 4*q2^4 + 4*q2^2*q3^2 - 4*q2^2 - 2*q3^2 + 1))/(4*q0^2*q1^2 + 4*q0^2*q2^2 + 4*q0^2*q3^2 + 4*q1^4 + 8*q1^2*q2^2 + 8*q1^2*q3^2 - 4*q1^2 + 4*q2^4 + 8*q2^2*q3^2 - 4*q2^2 + 4*q3^4 - 4*q3^2 + 1)^2,                                                                 (2*B_i3*(2*q0^2*q2 + 2*q1^2*q2 + 2*q2^3 + 6*q2*q3^2 - q2))/(4*q0^2*q1^2 + 4*q0^2*q2^2 + 4*q0^2*q3^2 + 4*q1^4 + 8*q1^2*q2^2 + 8*q1^2*q3^2 - 4*q1^2 + 4*q2^4 + 8*q2^2*q3^2 - 4*q2^2 + 4*q3^4 - 4*q3^2 + 1) - (B_i2*(- 8*q3*q2^2 + 4*q3))/(4*q0^2*q1^2 + 4*q0^2*q2^2 + 4*q0^2*q3^2 + 4*q1^4 + 8*q1^2*q2^2 + 8*q1^2*q3^2 - 4*q1^2 + 4*q2^4 + 8*q2^2*q3^2 - 4*q2^2 + 4*q3^4 - 4*q3^2 + 1) - (2*B_i1*(q0 - 4*q1*q2*q3))/(4*q0^2*q1^2 + 4*q0^2*q2^2 + 4*q0^2*q3^2 + 4*q1^4 + 8*q1^2*q2^2 + 8*q1^2*q3^2 - 4*q1^2 + 4*q2^4 + 8*q2^2*q3^2 - 4*q2^2 + 4*q3^4 - 4*q3^2 + 1) - (2*B_i1*(8*q0^2*q3 + 16*q1^2*q3 + 16*q2^2*q3 + 16*q3^3 - 8*q3)*(2*q0^2*q1*q2 - q0*q3 + 2*q1^3*q2 + 2*q1*q2^3 + 2*q1*q2*q3^2 - q1*q2))/(4*q0^2*q1^2 + 4*q0^2*q2^2 + 4*q0^2*q3^2 + 4*q1^4 + 8*q1^2*q2^2 + 8*q1^2*q3^2 - 4*q1^2 + 4*q2^4 + 8*q2^2*q3^2 - 4*q2^2 + 4*q3^4 - 4*q3^2 + 1)^2 - (2*B_i3*(8*q0^2*q3 + 16*q1^2*q3 + 16*q2^2*q3 + 16*q3^3 - 8*q3)*(2*q0^2*q2*q3 + q0*q1 + 2*q1^2*q2*q3 + 2*q2^3*q3 + 2*q2*q3^3 - q2*q3))/(4*q0^2*q1^2 + 4*q0^2*q2^2 + 4*q0^2*q3^2 + 4*q1^4 + 8*q1^2*q2^2 + 8*q1^2*q3^2 - 4*q1^2 + 4*q2^4 + 8*q2^2*q3^2 - 4*q2^2 + 4*q3^4 - 4*q3^2 + 1)^2 - (B_i2*(8*q0^2*q3 + 16*q1^2*q3 + 16*q2^2*q3 + 16*q3^3 - 8*q3)*(4*q0^2*q2^2 + 4*q1^2*q2^2 - 2*q1^2 + 4*q2^4 + 4*q2^2*q3^2 - 4*q2^2 - 2*q3^2 + 1))/(4*q0^2*q1^2 + 4*q0^2*q2^2 + 4*q0^2*q3^2 + 4*q1^4 + 8*q1^2*q2^2 + 8*q1^2*q3^2 - 4*q1^2 + 4*q2^4 + 8*q2^2*q3^2 - 4*q2^2 + 4*q3^4 - 4*q3^2 + 1)^2;
        (2*B_i1*(q2 + 4*q0*q1*q3))/(4*q0^2*q1^2 + 4*q0^2*q2^2 + 4*q0^2*q3^2 + 4*q1^4 + 8*q1^2*q2^2 + 8*q1^2*q3^2 - 4*q1^2 + 4*q2^4 + 8*q2^2*q3^2 - 4*q2^2 + 4*q3^4 - 4*q3^2 + 1) - (2*B_i2*(q1 - 4*q0*q2*q3))/(4*q0^2*q1^2 + 4*q0^2*q2^2 + 4*q0^2*q3^2 + 4*q1^4 + 8*q1^2*q2^2 + 8*q1^2*q3^2 - 4*q1^2 + 4*q2^4 + 8*q2^2*q3^2 - 4*q2^2 + 4*q3^4 - 4*q3^2 + 1) - (2*B_i1*(8*q0*q1^2 + 8*q0*q2^2 + 8*q0*q3^2)*(2*q0^2*q1*q3 + q0*q2 + 2*q1^3*q3 + 2*q1*q2^2*q3 + 2*q1*q3^3 - q1*q3))/(4*q0^2*q1^2 + 4*q0^2*q2^2 + 4*q0^2*q3^2 + 4*q1^4 + 8*q1^2*q2^2 + 8*q1^2*q3^2 - 4*q1^2 + 4*q2^4 + 8*q2^2*q3^2 - 4*q2^2 + 4*q3^4 - 4*q3^2 + 1)^2 - (2*B_i2*(8*q0*q1^2 + 8*q0*q2^2 + 8*q0*q3^2)*(2*q0^2*q2*q3 - q0*q1 + 2*q1^2*q2*q3 + 2*q2^3*q3 + 2*q2*q3^3 - q2*q3))/(4*q0^2*q1^2 + 4*q0^2*q2^2 + 4*q0^2*q3^2 + 4*q1^4 + 8*q1^2*q2^2 + 8*q1^2*q3^2 - 4*q1^2 + 4*q2^4 + 8*q2^2*q3^2 - 4*q2^2 + 4*q3^4 - 4*q3^2 + 1)^2 + (8*B_i3*q0*q3^2)/(4*q0^2*q1^2 + 4*q0^2*q2^2 + 4*q0^2*q3^2 + 4*q1^4 + 8*q1^2*q2^2 + 8*q1^2*q3^2 - 4*q1^2 + 4*q2^4 + 8*q2^2*q3^2 - 4*q2^2 + 4*q3^4 - 4*q3^2 + 1) - (B_i3*(8*q0*q1^2 + 8*q0*q2^2 + 8*q0*q3^2)*(4*q0^2*q3^2 + 4*q1^2*q3^2 - 2*q1^2 + 4*q2^2*q3^2 - 2*q2^2 + 4*q3^4 - 4*q3^2 + 1))/(4*q0^2*q1^2 + 4*q0^2*q2^2 + 4*q0^2*q3^2 + 4*q1^4 + 8*q1^2*q2^2 + 8*q1^2*q3^2 - 4*q1^2 + 4*q2^4 + 8*q2^2*q3^2 - 4*q2^2 + 4*q3^4 - 4*q3^2 + 1)^2,                                                                 (2*B_i1*(2*q0^2*q3 + 6*q1^2*q3 + 2*q2^2*q3 + 2*q3^3 - q3))/(4*q0^2*q1^2 + 4*q0^2*q2^2 + 4*q0^2*q3^2 + 4*q1^4 + 8*q1^2*q2^2 + 8*q1^2*q3^2 - 4*q1^2 + 4*q2^4 + 8*q2^2*q3^2 - 4*q2^2 + 4*q3^4 - 4*q3^2 + 1) - (B_i3*(- 8*q1*q3^2 + 4*q1))/(4*q0^2*q1^2 + 4*q0^2*q2^2 + 4*q0^2*q3^2 + 4*q1^4 + 8*q1^2*q2^2 + 8*q1^2*q3^2 - 4*q1^2 + 4*q2^4 + 8*q2^2*q3^2 - 4*q2^2 + 4*q3^4 - 4*q3^2 + 1) - (2*B_i2*(q0 - 4*q1*q2*q3))/(4*q0^2*q1^2 + 4*q0^2*q2^2 + 4*q0^2*q3^2 + 4*q1^4 + 8*q1^2*q2^2 + 8*q1^2*q3^2 - 4*q1^2 + 4*q2^4 + 8*q2^2*q3^2 - 4*q2^2 + 4*q3^4 - 4*q3^2 + 1) - (2*B_i1*(8*q0^2*q1 + 16*q1^3 + 16*q1*q2^2 + 16*q1*q3^2 - 8*q1)*(2*q0^2*q1*q3 + q0*q2 + 2*q1^3*q3 + 2*q1*q2^2*q3 + 2*q1*q3^3 - q1*q3))/(4*q0^2*q1^2 + 4*q0^2*q2^2 + 4*q0^2*q3^2 + 4*q1^4 + 8*q1^2*q2^2 + 8*q1^2*q3^2 - 4*q1^2 + 4*q2^4 + 8*q2^2*q3^2 - 4*q2^2 + 4*q3^4 - 4*q3^2 + 1)^2 - (2*B_i2*(8*q0^2*q1 + 16*q1^3 + 16*q1*q2^2 + 16*q1*q3^2 - 8*q1)*(2*q0^2*q2*q3 - q0*q1 + 2*q1^2*q2*q3 + 2*q2^3*q3 + 2*q2*q3^3 - q2*q3))/(4*q0^2*q1^2 + 4*q0^2*q2^2 + 4*q0^2*q3^2 + 4*q1^4 + 8*q1^2*q2^2 + 8*q1^2*q3^2 - 4*q1^2 + 4*q2^4 + 8*q2^2*q3^2 - 4*q2^2 + 4*q3^4 - 4*q3^2 + 1)^2 - (B_i3*(8*q0^2*q1 + 16*q1^3 + 16*q1*q2^2 + 16*q1*q3^2 - 8*q1)*(4*q0^2*q3^2 + 4*q1^2*q3^2 - 2*q1^2 + 4*q2^2*q3^2 - 2*q2^2 + 4*q3^4 - 4*q3^2 + 1))/(4*q0^2*q1^2 + 4*q0^2*q2^2 + 4*q0^2*q3^2 + 4*q1^4 + 8*q1^2*q2^2 + 8*q1^2*q3^2 - 4*q1^2 + 4*q2^4 + 8*q2^2*q3^2 - 4*q2^2 + 4*q3^4 - 4*q3^2 + 1)^2,                                                                 (2*B_i1*(q0 + 4*q1*q2*q3))/(4*q0^2*q1^2 + 4*q0^2*q2^2 + 4*q0^2*q3^2 + 4*q1^4 + 8*q1^2*q2^2 + 8*q1^2*q3^2 - 4*q1^2 + 4*q2^4 + 8*q2^2*q3^2 - 4*q2^2 + 4*q3^4 - 4*q3^2 + 1) - (B_i3*(- 8*q2*q3^2 + 4*q2))/(4*q0^2*q1^2 + 4*q0^2*q2^2 + 4*q0^2*q3^2 + 4*q1^4 + 8*q1^2*q2^2 + 8*q1^2*q3^2 - 4*q1^2 + 4*q2^4 + 8*q2^2*q3^2 - 4*q2^2 + 4*q3^4 - 4*q3^2 + 1) + (2*B_i2*(2*q0^2*q3 + 2*q1^2*q3 + 6*q2^2*q3 + 2*q3^3 - q3))/(4*q0^2*q1^2 + 4*q0^2*q2^2 + 4*q0^2*q3^2 + 4*q1^4 + 8*q1^2*q2^2 + 8*q1^2*q3^2 - 4*q1^2 + 4*q2^4 + 8*q2^2*q3^2 - 4*q2^2 + 4*q3^4 - 4*q3^2 + 1) - (2*B_i1*(8*q0^2*q2 + 16*q1^2*q2 + 16*q2^3 + 16*q2*q3^2 - 8*q2)*(2*q0^2*q1*q3 + q0*q2 + 2*q1^3*q3 + 2*q1*q2^2*q3 + 2*q1*q3^3 - q1*q3))/(4*q0^2*q1^2 + 4*q0^2*q2^2 + 4*q0^2*q3^2 + 4*q1^4 + 8*q1^2*q2^2 + 8*q1^2*q3^2 - 4*q1^2 + 4*q2^4 + 8*q2^2*q3^2 - 4*q2^2 + 4*q3^4 - 4*q3^2 + 1)^2 - (2*B_i2*(8*q0^2*q2 + 16*q1^2*q2 + 16*q2^3 + 16*q2*q3^2 - 8*q2)*(2*q0^2*q2*q3 - q0*q1 + 2*q1^2*q2*q3 + 2*q2^3*q3 + 2*q2*q3^3 - q2*q3))/(4*q0^2*q1^2 + 4*q0^2*q2^2 + 4*q0^2*q3^2 + 4*q1^4 + 8*q1^2*q2^2 + 8*q1^2*q3^2 - 4*q1^2 + 4*q2^4 + 8*q2^2*q3^2 - 4*q2^2 + 4*q3^4 - 4*q3^2 + 1)^2 - (B_i3*(8*q0^2*q2 + 16*q1^2*q2 + 16*q2^3 + 16*q2*q3^2 - 8*q2)*(4*q0^2*q3^2 + 4*q1^2*q3^2 - 2*q1^2 + 4*q2^2*q3^2 - 2*q2^2 + 4*q3^4 - 4*q3^2 + 1))/(4*q0^2*q1^2 + 4*q0^2*q2^2 + 4*q0^2*q3^2 + 4*q1^4 + 8*q1^2*q2^2 + 8*q1^2*q3^2 - 4*q1^2 + 4*q2^4 + 8*q2^2*q3^2 - 4*q2^2 + 4*q3^4 - 4*q3^2 + 1)^2, (2*B_i1*(2*q0^2*q1 + 2*q1^3 + 2*q1*q2^2 + 6*q1*q3^2 - q1))/(4*q0^2*q1^2 + 4*q0^2*q2^2 + 4*q0^2*q3^2 + 4*q1^4 + 8*q1^2*q2^2 + 8*q1^2*q3^2 - 4*q1^2 + 4*q2^4 + 8*q2^2*q3^2 - 4*q2^2 + 4*q3^4 - 4*q3^2 + 1) + (2*B_i2*(2*q0^2*q2 + 2*q1^2*q2 + 2*q2^3 + 6*q2*q3^2 - q2))/(4*q0^2*q1^2 + 4*q0^2*q2^2 + 4*q0^2*q3^2 + 4*q1^4 + 8*q1^2*q2^2 + 8*q1^2*q3^2 - 4*q1^2 + 4*q2^4 + 8*q2^2*q3^2 - 4*q2^2 + 4*q3^4 - 4*q3^2 + 1) + (B_i3*(8*q0^2*q3 + 8*q1^2*q3 + 8*q2^2*q3 + 16*q3^3 - 8*q3))/(4*q0^2*q1^2 + 4*q0^2*q2^2 + 4*q0^2*q3^2 + 4*q1^4 + 8*q1^2*q2^2 + 8*q1^2*q3^2 - 4*q1^2 + 4*q2^4 + 8*q2^2*q3^2 - 4*q2^2 + 4*q3^4 - 4*q3^2 + 1) - (2*B_i1*(8*q0^2*q3 + 16*q1^2*q3 + 16*q2^2*q3 + 16*q3^3 - 8*q3)*(2*q0^2*q1*q3 + q0*q2 + 2*q1^3*q3 + 2*q1*q2^2*q3 + 2*q1*q3^3 - q1*q3))/(4*q0^2*q1^2 + 4*q0^2*q2^2 + 4*q0^2*q3^2 + 4*q1^4 + 8*q1^2*q2^2 + 8*q1^2*q3^2 - 4*q1^2 + 4*q2^4 + 8*q2^2*q3^2 - 4*q2^2 + 4*q3^4 - 4*q3^2 + 1)^2 - (2*B_i2*(8*q0^2*q3 + 16*q1^2*q3 + 16*q2^2*q3 + 16*q3^3 - 8*q3)*(2*q0^2*q2*q3 - q0*q1 + 2*q1^2*q2*q3 + 2*q2^3*q3 + 2*q2*q3^3 - q2*q3))/(4*q0^2*q1^2 + 4*q0^2*q2^2 + 4*q0^2*q3^2 + 4*q1^4 + 8*q1^2*q2^2 + 8*q1^2*q3^2 - 4*q1^2 + 4*q2^4 + 8*q2^2*q3^2 - 4*q2^2 + 4*q3^4 - 4*q3^2 + 1)^2 - (B_i3*(8*q0^2*q3 + 16*q1^2*q3 + 16*q2^2*q3 + 16*q3^3 - 8*q3)*(4*q0^2*q3^2 + 4*q1^2*q3^2 - 2*q1^2 + 4*q2^2*q3^2 - 2*q2^2 + 4*q3^4 - 4*q3^2 + 1))/(4*q0^2*q1^2 + 4*q0^2*q2^2 + 4*q0^2*q3^2 + 4*q1^4 + 8*q1^2*q2^2 + 8*q1^2*q3^2 - 4*q1^2 + 4*q2^4 + 8*q2^2*q3^2 - 4*q2^2 + 4*q3^4 - 4*q3^2 + 1)^2];
dh3dd = zeros(3,3);

%dim=9x12           
dhdX = [dh1dx dh1dvr dh1dq dh1dd;
        dh2dx dh2dvr dh2dq dh2dd;
        dh3dx dh3dvr dh3dq dh3dd;];
end

% %% quaternion library
% function new_D=quat_D(q,D)
%       q0=q(1);
%       qv=q(2:4);
%       R=eye(3)+2*q0*hat(qv)+2*hat(qv)*hat(qv);
%       new_D=R*D*R';
% end
% 
% function vec=quat_v(q,v,type)
%     if type == 0 %q*v*q^-1
%       q0=q(1);
%       qv=q(2:4);
%       R=eye(3)+2*q0*hat(qv)+2*hat(qv)*hat(qv);
%       vec=R*v;
%     elseif type == 1 %q^-1*v*q
%       q0=q(1);
%       qv=q(2:4);
%       R=eye(3)+2*q0*hat(qv)+2*hat(qv)*hat(qv);
%       vec=inv(R)*v;
%     end
% end
